simulink model "SeaPort"  (R2023b)
settings: Solver=VariableStepAuto  StartTime=0.0  StopTime=2.0  RelTol=1e-3
(part 1 of 3)
settings Model: Creator=Stefano  LastModifiedBy=stefanopanzieri
settings SolverCC: AlgebraicLoopSolver=TrustRegion
settings OptimizationCC: ReuseModelBlockBuffer=off
settings DebuggingCC: UnconnectedInputMsg=warning  UnconnectedOutputMsg=warning  UnconnectedLineMsg=warning
settings ModelReferenceCC: EnableRefExpFcnMdlSchedulingChecks=on
settings SFSimCC: CustomCodeUndefinedFunction=UseInterfaceOnly
settings RTWCC: DLArmComputeVersion=19.05

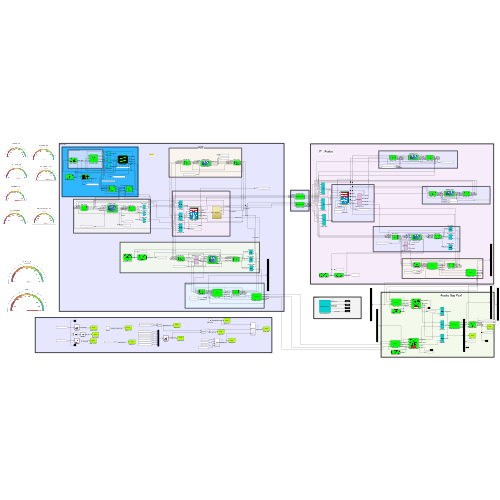
[thumbnail: Simulink's stored preview of the top-level diagram]
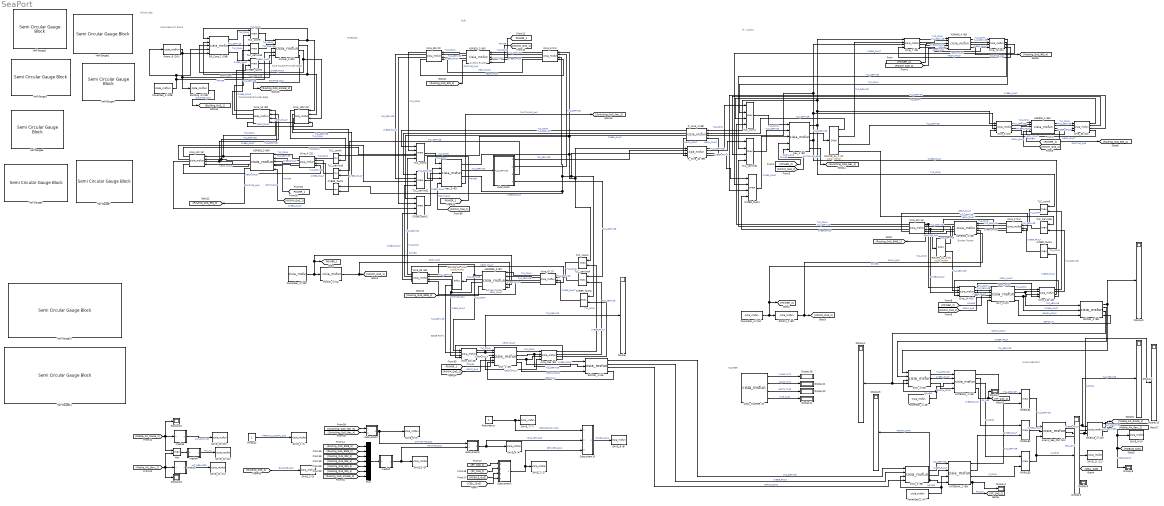
== system SeaPort ==
  note: EDGE POP 1
  note: IT - Aveiro
  note: Altice Labs
  note: CORE DC
  note: Border Router
  note: Access Router
  note: Core Router/Provider Edge
  note: ALB
  note: Aveiro Sea Port
  note: Border Router
  note: Core Network Room
  note: Core Router/Provider Edge
  note: MASTER
  5G_Core_1 (198) : M-S-Function  FunctionName=cisia_msfun  Parameters=Parameter1, Parameter2, Parameter3, resources, Parameter10, codeupdate, step_received, step_computed, dynamic_computed, step_sended, id_entity, id_project, id_type, name_type, color  mask(S-function:msfcn_unit_delay){Parameter1='5G_Core_1', Parameter2=1, Parameter3='ORO', resources=*** INPUT RESOURCES *** NUM_INPUTS 5 TLC_CONN (20) TLC_SERVICE (20) CYBER_FAULT (10) POWER (1) ROOM_QoS (1)  *** STATE VARIABLES *** NUM_VARIABLES 22 Operative_Level(NUMERIC)(1)(1) TLC_services(NUMERIC_ARRAY)(20)(0  0  0  0  0  0  1  1  0  0  0  0  0  0  0  0  0  0  0  0) TLC_service_names(STRING)(100)(5G_CU_DU_SLICE) Connection(NUMERIC_ARRAY)(20)(0  0  0  0  0  0  1  1  0  0  0  0  0  0  0  0  0  0  0  0) Dos_attack(NUMERIC)(1)(0) MITM_attack(NUMERIC)(1)(0) Virus_Attack(NUMERIC)(1)(0) Port_Scan_Attack(NUMERIC)(1)(0) Cyber_Fault(NUMERIC_ARRAY)(10)(0  0  0  0  0  0  0  0  0  0) BGP_hijacking(NUMERIC)(1)(0) Mechanical_Fault(NUMERIC)(1)(0) Conn_Fault(NUMERIC)(1)(0) Consumed_Services(NUMERIC_ARRAY)(20)(0  0  0  0  0  0  0  0  0  0  0  0  0  0  0  0  0  0  0  0) Service_Fault(NUMERIC)(1)(0) Redundancy_Fault(NUMERIC)(1)(0) BotNet_Attack(NUMERIC)(1)(0) Data_Corruption(NUMERIC)(1)(0) syslog_adm_login(NUMERIC)(1)(0) SW_Change(NUMERIC)(1)(0) Config_Change(NUMERIC)(1)(0) Port_Saturation(NUMERIC)(1)(0) TLC_revoke(NUMERIC_ARRAY)(20)(0  0  0  0  0  0  0  0  0  0  0  0  0  0  0  0  0  0  0  0)  *** OUTPUT RESOURCES *** NUM_OUTPUTS 3 TLC_CONN (20) TLC_SERVICE (20) CYBER_FAULT (10), Parameter10=off, codeupdate=off, step_received=Connection=max(Connection_init,TLC_CONN); TLC_services=max(TLC_services_init,TLC_SERVICE); TLC_services=mod(TLC_services,10); TLC_revoke=floor(TLC_SERVICE/10); Mechanical_Fault=max([Mechanical_Fault Mechanical_Fault_init]);  Cyber_Fault=max(CYBER_FAULT, transpose([Dos_attack   MITM_attack Virus_Attack Port_Scan_Attack  BGP_hijacking BotNet_Attack Data_Corruption SW_Change Config_Change Port_Saturation]));    %if (cisia.major_time)>=2    %Dos_attack=1;    %TLC_services(5)=0;   %TLC_revoke(5)=1; %end    Conn_Fault=max([Dos_attack  Mechanical_Fault  1-POWER 1-ROOM_QoS] );  Service_Fault=max(abs(Consumed_Services.*TLC_services-Consumed_Services)); Redundancy_Fault=max(abs(Consumed_Services.*TLC_CONN-Consumed_Services));  Operative_Level=(1-Conn_Fault)*(1-0.5*max(Cyber_Fault))*(1-Service_Fault);, step_computed=, dynamic_computed=, step_sended=TLC_CONN=Connection*(1-Conn_Fault); TLC_SERVICE=TLC_services*(1-Conn_Fault)*(1-Service_Fault)*(1 -syslog_adm_login)+10*TLC_revoke; %TLC_SERVICE=TLC_services CYBER_FAULT=Cyber_Fault*(1-Conn_Fault);, id_entity=198, id_project=40, id_type=38, name_type=5G_Core, color=#E7A6FF}
      mask prompts: Parameter1 "entity name"; Parameter2 "sampling time"; Parameter3 "project"; resources "input resources and state variables"; Parameter10 "Bring state variables to output"; codeupdate "update code from mask"
      mask help: This is a level-2 MATLAB file S-function which demonstrates CISIA entity
      mask DialogControl Container1 Prompt: All parameters
      mask Display: image('Icons/5G_Core.png')
  ANTENNA_1 (56) : M-S-Function  FunctionName=cisia_msfun  Parameters=Parameter1, Parameter2, Parameter3, resources, Parameter10, codeupdate, step_received, step_computed, dynamic_computed, step_sended, id_entity, id_project, id_type, name_type, color  mask(S-function:msfcn_unit_delay){Parameter1='ANTENNA_1', Parameter2=1, Parameter3='ORO', resources=*** INPUT RESOURCES *** NUM_INPUTS 4 TLC_SERVICE (20) CYBER_FAULT (10) POWER (1) NGPON_CONN (20)  *** STATE VARIABLES *** NUM_VARIABLES 20 Operative_Level(NUMERIC)(1)(1) TLC_services(NUMERIC_ARRAY)(20)(0  0  0  0  0  0  0  0  0  0  0  0  0  0  0  0  0  0  0  0) Connection(NUMERIC_ARRAY)(20)(0  0  0  0  0  0  0  0  0  0  0  0  0  0  0  0  0  0  0  0) Dos_attack(NUMERIC)(1)(0) MITM_attack(NUMERIC)(1)(0) Virus_Attack(NUMERIC)(1)(0) Port_Scan_Attack(NUMERIC)(1)(0) Cyber_Fault(NUMERIC_ARRAY)(10)(0  0  0  0  0  0  0  0  0  0) MyConn(NUMERIC_ARRAY)(20)(0  0  0  0  0  0  0  0  0  0  0  0  0  0  0  0  0  0  0  0) BGP_hijacking(NUMERIC)(1)(0) Mechanical_Fault(NUMERIC)(1)(0) Conn_Fault(NUMERIC)(1)(0) Consumed_Services(NUMERIC_ARRAY)(20)(0  0  0  0  0  0  1  0  0  0  0  0  0  0  0  0  0  0  0  0) BotNet_Attack(NUMERIC)(1)(0) Data_Corruption(NUMERIC)(1)(0) SW_Change(NUMERIC)(1)(0) Config_Change(NUMERIC)(1)(0) Port_Saturation(NUMERIC)(1)(0) My_Service(NUMERIC)(1)(0) TLC_revoke(NUMERIC_ARRAY)(20)(0  0  0  0  0  0  0  0  0  0  0  0  0  0  0  0  0  0  0  0)  *** OUTPUT RESOURCES *** NUM_OUTPUTS 4 TLC_SERVICE (20) CYBER_FAULT (10) R_CONN (20) RF_QoS (1), Parameter10=off, codeupdate=off, step_received=Connection=max(Connection_init,NGPON_CONN); TLC_services=max(TLC_services_init,TLC_SERVICE); TLC_services=mod(TLC_services,10); TLC_revoke=floor(TLC_SERVICE/10);  Cyber_Fault=max(CYBER_FAULT, transpose([Dos_attack   MITM_attack Virus_Attack Port_Scan_Attack  BGP_hijacking BotNet_Attack Data_Corruption SW_Change Config_Change Port_Saturation]));  % Vale 1 in presenza di fault Conn_Fault=max([Dos_attack  Mechanical_Fault  1-POWER] );  Service_Fault=max(abs(Consumed_Services.*TLC_services-Consumed_Services)); Redundancy_Fault=max(abs(Consumed_Services.*NGPON_CONN-Consumed_Services));   Operative_Level=(1-Conn_Fault)*max(max(NGPON_CONN),0.5)*((2*(1-Service_Fault)+(1-Redundancy_Fault))/3);  % Il servizio utilizzato My_Service=max([(1-Service_Fault) (1-Redundancy_Fault)/2]);, step_computed=, dynamic_computed=, step_sended=R_CONN=Connection*(1-Conn_Fault); TLC_SERVICE=TLC_services*(1-Conn_Fault)+10*TLC_revoke;  Cyber_Transmitted=min(Cyber_Fault, transpose([0 0 1 0 1 1 0 0 0 1])); CYBER_FAULT=Cyber_Transmitted*(1-Conn_Fault);   RF_QoS=My_Service;, id_entity=56, id_project=40, id_type=13, name_type=RU-DU_ANTENNA, color=#90DB5A}
      mask prompts: Parameter1 "entity name"; Parameter2 "sampling time"; Parameter3 "project"; resources "input resources and state variables"; Parameter10 "Bring state variables to output"; codeupdate "update code from mask"
      mask help: This is a level-2 MATLAB file S-function which demonstrates CISIA entity
      mask DialogControl Container1 Prompt: All parameters
      mask Display: image('Icons/RU-DU_ANTENNA.png')
  ANTENNA_2 (60) : M-S-Function  FunctionName=cisia_msfun  Parameters=Parameter1, Parameter2, Parameter3, resources, Parameter10, codeupdate, step_received, step_computed, dynamic_computed, step_sended, id_entity, id_project, id_type, name_type, color  mask(S-function:msfcn_unit_delay){Parameter1='ANTENNA_2', Parameter2=1, Parameter3='ORO', resources=*** INPUT RESOURCES *** NUM_INPUTS 4 TLC_SERVICE (20) CYBER_FAULT (10) POWER (1) NGPON_CONN (20)  *** STATE VARIABLES *** NUM_VARIABLES 20 Operative_Level(NUMERIC)(1)(1) TLC_services(NUMERIC_ARRAY)(20)(0  0  0  0  0  0  0  0  0  0  0  0  0  0  0  0  0  0  0  0) Connection(NUMERIC_ARRAY)(20)(0  0  0  0  0  0  0  0  0  0  0  0  0  0  0  0  0  0  0  0) Dos_attack(NUMERIC)(1)(0) MITM_attack(NUMERIC)(1)(0) Virus_Attack(NUMERIC)(1)(0) Port_Scan_Attack(NUMERIC)(1)(0) Cyber_Fault(NUMERIC_ARRAY)(10)(0  0  0  0  0  0  0  0  0  0) MyConn(NUMERIC_ARRAY)(20)(0  0  0  0  0  0  0  0  0  0  0  0  0  0  0  0  0  0  0  0) BGP_hijacking(NUMERIC)(1)(0) Mechanical_Fault(NUMERIC)(1)(0) Conn_Fault(NUMERIC)(1)(0) Consumed_Services(NUMERIC_ARRAY)(20)(0  0  0  0  0  0  1  0  0  0  0  0  0  0  0  0  0  0  0  0) BotNet_Attack(NUMERIC)(1)(0) Data_Corruption(NUMERIC)(1)(0) SW_Change(NUMERIC)(1)(0) Config_Change(NUMERIC)(1)(0) Port_Saturation(NUMERIC)(1)(0) My_Service(NUMERIC)(1)(0) TLC_revoke(NUMERIC_ARRAY)(20)(0  0  0  0  0  0  0  0  0  0  0  0  0  0  0  0  0  0  0  0)  *** OUTPUT RESOURCES *** NUM_OUTPUTS 4 TLC_SERVICE (20) CYBER_FAULT (10) R_CONN (20) RF_QoS (1), Parameter10=off, codeupdate=off, step_received=Connection=max(Connection_init,NGPON_CONN); TLC_services=max(TLC_services_init,TLC_SERVICE); TLC_services=mod(TLC_services,10); TLC_revoke=floor(TLC_SERVICE/10);  Cyber_Fault=max(CYBER_FAULT, transpose([Dos_attack   MITM_attack Virus_Attack Port_Scan_Attack  BGP_hijacking BotNet_Attack Data_Corruption SW_Change Config_Change Port_Saturation]));  % Vale 1 in presenza di fault Conn_Fault=max([Dos_attack  Mechanical_Fault  1-POWER] );  Service_Fault=max(abs(Consumed_Services.*TLC_services-Consumed_Services)); Redundancy_Fault=max(abs(Consumed_Services.*NGPON_CONN-Consumed_Services));   Operative_Level=(1-Conn_Fault)*max(max(NGPON_CONN),0.5)*((2*(1-Service_Fault)+(1-Redundancy_Fault))/3);  % Il servizio utilizzato My_Service=max([(1-Service_Fault) (1-Redundancy_Fault)/2]);, step_computed=, dynamic_computed=, step_sended=R_CONN=Connection*(1-Conn_Fault); TLC_SERVICE=TLC_services*(1-Conn_Fault)+10*TLC_revoke;  Cyber_Transmitted=min(Cyber_Fault, transpose([0 0 1 0 1 1 0 0 0 1])); CYBER_FAULT=Cyber_Transmitted*(1-Conn_Fault);   RF_QoS=My_Service;, id_entity=60, id_project=40, id_type=13, name_type=RU-DU_ANTENNA, color=#90DB5A}
      mask prompts: Parameter1 "entity name"; Parameter2 "sampling time"; Parameter3 "project"; resources "input resources and state variables"; Parameter10 "Bring state variables to output"; codeupdate "update code from mask"
      mask help: This is a level-2 MATLAB file S-function which demonstrates CISIA entity
      mask DialogControl Container1 Prompt: All parameters
      mask Display: image('Icons/RU-DU_ANTENNA.png')
  ASR9006_3 (87) : M-S-Function  FunctionName=cisia_msfun  Parameters=Parameter1, Parameter2, Parameter3, resources, Parameter10, codeupdate, step_received, step_computed, dynamic_computed, step_sended, id_entity, id_project, id_type, name_type, color  mask(S-function:msfcn_unit_delay){Parameter1='ASR9006_3', Parameter2=1, Parameter3='ORO', resources=*** INPUT RESOURCES *** NUM_INPUTS 5 TLC_CONN (20) TLC_SERVICE (20) CYBER_FAULT (10) POWER (1) ROOM_QoS (1)  *** STATE VARIABLES *** NUM_VARIABLES 26 Operative_Level(NUMERIC)(1)(1) TLC_services(NUMERIC_ARRAY)(20)(0  0  0  0  0  0  0  0  0  0  0  0  0  0  0  0  0  0  0  0) TLC_service_names(STRING)(100)() Connection(NUMERIC_ARRAY)(20)(0  0  0  0  0  0  0  0  0  0  0  0  0  0  0  0  0  0  0  0) Dos_attack(NUMERIC)(1)(0) MITM_attack(NUMERIC)(1)(0) Virus_Attack(NUMERIC)(1)(0) Port_Scan_Attack(NUMERIC)(1)(0) Cyber_Fault(NUMERIC_ARRAY)(10)(0  0  0  0  0  0  0  0  0  0) BGP_hijacking(NUMERIC)(1)(0) Mechanical_Fault(NUMERIC)(1)(0) Flooding_Fault(NUMERIC)(1)(0) OutboundQoS(NUMERIC)(1)(0) Conn_Fault(NUMERIC)(1)(0) BotNet_Attack(NUMERIC)(1)(0) Data_Corruption(NUMERIC)(1)(0) syslog_adm_login(NUMERIC)(1)(0) SW_Change(NUMERIC)(1)(0) Config_Change(NUMERIC)(1)(0) Port_Saturation(NUMERIC)(1)(0) Congestion_Fault(NUMERIC)(1)(0) Earthquake_Fault(NUMERIC)(1)(0) TLC_revoke(NUMERIC_ARRAY)(20)(0  0  0  0  0  0  0  0  0  0  0  0  0  0  0  0  0  0  0  0) Room_Fault(NUMERIC)(1)(0) Route_Poisoning(NUMERIC)(1)(0) Interface_Down(NUMERIC)(1)(0)  *** OUTPUT RESOURCES *** NUM_OUTPUTS 4 TLC_CONN (20) TLC_SERVICE (20) CYBER_FAULT (10) ROUTING_QoS (1), Parameter10=off, codeupdate=off, step_received=Connection=max(Connection_init,TLC_CONN); TLC_services=max(TLC_services_init,TLC_SERVICE); TLC_services=mod(TLC_services,10); TLC_revoke=floor(TLC_SERVICE/10);  Cyber_Fault=max(CYBER_FAULT, transpose([Dos_attack   MITM_attack Virus_Attack Port_Scan_Attack  BGP_hijacking BotNet_Attack Data_Corruption SW_Change Config_Change Port_Saturation]));   Conn_Fault=max([Dos_attack BGP_hijacking Route_Poisoning Interface_Down Mechanical_Fault  1-POWER 1-ROOM_QoS Earthquake_Fault] );  Room_Fault=1-ROOM_QoS;  Operative_Level=(1-Room_Fault)*(1-Conn_Fault)*max(max(TLC_services),0.5)*(1-0.5*max(Cyber_Fault));, step_computed=, dynamic_computed=, step_sended=TLC_CONN=Connection*(1-Conn_Fault); TLC_SERVICE=TLC_services*(1-Room_Fault)*(1-Conn_Fault)*(1-syslog_adm_login)+10*TLC_revoke;   Cyber_Transmitted=min(Cyber_Fault, transpose([0 0 1 0 1 1 0 0 0 1]));  CYBER_FAULT=Cyber_Transmitted*(1-Conn_Fault);  ROUTING_QoS=Operative_Level;, id_entity=87, id_project=40, id_type=3, name_type=CISCO_router, color=#4DBEEE}
      mask prompts: Parameter1 "entity name"; Parameter2 "sampling time"; Parameter3 "project"; resources "input resources and state variables"; Parameter10 "Bring state variables to output"; codeupdate "update code from mask"
      mask help: This is a level-2 MATLAB file S-function which demonstrates CISIA entity
      mask DialogControl Container1 Prompt: All parameters
      mask Display: image('Icons/CISCO_router.png')
  ASR9006_4 (88) : M-S-Function  FunctionName=cisia_msfun  Parameters=Parameter1, Parameter2, Parameter3, resources, Parameter10, codeupdate, step_received, step_computed, dynamic_computed, step_sended, id_entity, id_project, id_type, name_type, color  mask(S-function:msfcn_unit_delay){Parameter1='ASR9006_4', Parameter2=1, Parameter3='ORO', resources=*** INPUT RESOURCES *** NUM_INPUTS 5 TLC_CONN (20) TLC_SERVICE (20) CYBER_FAULT (10) POWER (1) ROOM_QoS (1)  *** STATE VARIABLES *** NUM_VARIABLES 26 Operative_Level(NUMERIC)(1)(1) TLC_services(NUMERIC_ARRAY)(20)(0  0  0  0  0  0  0  0  0  0  0  0  0  0  0  0  0  0  0  0) TLC_service_names(STRING)(100)() Connection(NUMERIC_ARRAY)(20)(0  0  0  0  0  0  0  0  0  0  0  0  0  0  0  0  0  0  0  0) Dos_attack(NUMERIC)(1)(0) MITM_attack(NUMERIC)(1)(0) Virus_Attack(NUMERIC)(1)(0) Port_Scan_Attack(NUMERIC)(1)(0) Cyber_Fault(NUMERIC_ARRAY)(10)(0  0  0  0  0  0  0  0  0  0) BGP_hijacking(NUMERIC)(1)(0) Mechanical_Fault(NUMERIC)(1)(0) Flooding_Fault(NUMERIC)(1)(0) OutboundQoS(NUMERIC)(1)(0) Conn_Fault(NUMERIC)(1)(0) BotNet_Attack(NUMERIC)(1)(0) Data_Corruption(NUMERIC)(1)(0) syslog_adm_login(NUMERIC)(1)(0) SW_Change(NUMERIC)(1)(0) Config_Change(NUMERIC)(1)(0) Port_Saturation(NUMERIC)(1)(0) Congestion_Fault(NUMERIC)(1)(0) Earthquake_Fault(NUMERIC)(1)(0) TLC_revoke(NUMERIC_ARRAY)(20)(0  0  0  0  0  0  0  0  0  0  0  0  0  0  0  0  0  0  0  0) Room_Fault(NUMERIC)(1)(0) Route_Poisoning(NUMERIC)(1)(0) Interface_Down(NUMERIC)(1)(0)  *** OUTPUT RESOURCES *** NUM_OUTPUTS 4 TLC_CONN (20) TLC_SERVICE (20) CYBER_FAULT (10) ROUTING_QoS (1), Parameter10=off, codeupdate=off, step_received=Connection=max(Connection_init,TLC_CONN); TLC_services=max(TLC_services_init,TLC_SERVICE); TLC_services=mod(TLC_services,10); TLC_revoke=floor(TLC_SERVICE/10);  Cyber_Fault=max(CYBER_FAULT, transpose([Dos_attack   MITM_attack Virus_Attack Port_Scan_Attack  BGP_hijacking BotNet_Attack Data_Corruption SW_Change Config_Change Port_Saturation]));   Conn_Fault=max([Dos_attack BGP_hijacking Route_Poisoning Interface_Down Mechanical_Fault  1-POWER 1-ROOM_QoS Earthquake_Fault] );  Room_Fault=1-ROOM_QoS;  Operative_Level=(1-Room_Fault)*(1-Conn_Fault)*max(max(TLC_services),0.5)*(1-0.5*max(Cyber_Fault));, step_computed=, dynamic_computed=, step_sended=TLC_CONN=Connection*(1-Conn_Fault); TLC_SERVICE=TLC_services*(1-Room_Fault)*(1-Conn_Fault)*(1-syslog_adm_login)+10*TLC_revoke;   Cyber_Transmitted=min(Cyber_Fault, transpose([0 0 1 0 1 1 0 0 0 1]));  CYBER_FAULT=Cyber_Transmitted*(1-Conn_Fault);  ROUTING_QoS=Operative_Level;, id_entity=88, id_project=40, id_type=3, name_type=CISCO_router, color=#4DBEEE}
      mask prompts: Parameter1 "entity name"; Parameter2 "sampling time"; Parameter3 "project"; resources "input resources and state variables"; Parameter10 "Bring state variables to output"; codeupdate "update code from mask"
      mask help: This is a level-2 MATLAB file S-function which demonstrates CISIA entity
      mask DialogControl Container1 Prompt: All parameters
      mask Display: image('Icons/CISCO_router.png')
  ASR903_3 (89) : M-S-Function  FunctionName=cisia_msfun  Parameters=Parameter1, Parameter2, Parameter3, resources, Parameter10, codeupdate, step_received, step_computed, dynamic_computed, step_sended, id_entity, id_project, id_type, name_type, color  mask(S-function:msfcn_unit_delay){Parameter1='ASR903_3', Parameter2=1, Parameter3='ORO', resources=*** INPUT RESOURCES *** NUM_INPUTS 5 TLC_CONN (20) TLC_SERVICE (20) CYBER_FAULT (10) POWER (1) ROOM_QoS (1)  *** STATE VARIABLES *** NUM_VARIABLES 26 Operative_Level(NUMERIC)(1)(1) TLC_services(NUMERIC_ARRAY)(20)(0  0  0  0  0  0  0  0  0  0  0  0  0  0  0  0  0  0  0  0) TLC_service_names(STRING)(100)() Connection(NUMERIC_ARRAY)(20)(0  0  0  0  0  0  0  0  0  0  0  0  0  0  0  0  0  0  0  0) Dos_attack(NUMERIC)(1)(0) MITM_attack(NUMERIC)(1)(0) Virus_Attack(NUMERIC)(1)(0) Port_Scan_Attack(NUMERIC)(1)(0) Cyber_Fault(NUMERIC_ARRAY)(10)(0  0  0  0  0  0  0  0  0  0) BGP_hijacking(NUMERIC)(1)(0) Mechanical_Fault(NUMERIC)(1)(0) Flooding_Fault(NUMERIC)(1)(0) OutboundQoS(NUMERIC)(1)(0) Conn_Fault(NUMERIC)(1)(0) BotNet_Attack(NUMERIC)(1)(0) Data_Corruption(NUMERIC)(1)(0) syslog_adm_login(NUMERIC)(1)(0) SW_Change(NUMERIC)(1)(0) Config_Change(NUMERIC)(1)(0) Port_Saturation(NUMERIC)(1)(0) Congestion_Fault(NUMERIC)(1)(0) Earthquake_Fault(NUMERIC)(1)(0) TLC_revoke(NUMERIC_ARRAY)(20)(0  0  0  0  0  0  0  0  0  0  0  0  0  0  0  0  0  0  0  0) Room_Fault(NUMERIC)(1)(0) Route_Poisoning(NUMERIC)(1)(0) Interface_Down(NUMERIC)(1)(0)  *** OUTPUT RESOURCES *** NUM_OUTPUTS 4 TLC_CONN (20) TLC_SERVICE (20) CYBER_FAULT (10) ROUTING_QoS (1), Parameter10=off, codeupdate=off, step_received=Connection=max(Connection_init,TLC_CONN); TLC_services=max(TLC_services_init,TLC_SERVICE); TLC_services=mod(TLC_services,10); TLC_revoke=floor(TLC_SERVICE/10);  Cyber_Fault=max(CYBER_FAULT, transpose([Dos_attack   MITM_attack Virus_Attack Port_Scan_Attack  BGP_hijacking BotNet_Attack Data_Corruption SW_Change Config_Change Port_Saturation]));   Conn_Fault=max([Dos_attack BGP_hijacking Route_Poisoning Interface_Down Mechanical_Fault  1-POWER 1-ROOM_QoS Earthquake_Fault] );  Room_Fault=1-ROOM_QoS;  Operative_Level=(1-Room_Fault)*(1-Conn_Fault)*max(max(TLC_services),0.5)*(1-0.5*max(Cyber_Fault));, step_computed=, dynamic_computed=, step_sended=TLC_CONN=Connection*(1-Conn_Fault); TLC_SERVICE=TLC_services*(1-Room_Fault)*(1-Conn_Fault)*(1-syslog_adm_login)+10*TLC_revoke;   Cyber_Transmitted=min(Cyber_Fault, transpose([0 0 1 0 1 1 0 0 0 1]));  CYBER_FAULT=Cyber_Transmitted*(1-Conn_Fault);  ROUTING_QoS=Operative_Level;, id_entity=89, id_project=40, id_type=3, name_type=CISCO_router, color=#4DBEEE}
      mask prompts: Parameter1 "entity name"; Parameter2 "sampling time"; Parameter3 "project"; resources "input resources and state variables"; Parameter10 "Bring state variables to output"; codeupdate "update code from mask"
      mask help: This is a level-2 MATLAB file S-function which demonstrates CISIA entity
      mask DialogControl Container1 Prompt: All parameters
      mask Display: image('Icons/CISCO_router.png')
  ASR903_4 (90) : M-S-Function  FunctionName=cisia_msfun  Parameters=Parameter1, Parameter2, Parameter3, resources, Parameter10, codeupdate, step_received, step_computed, dynamic_computed, step_sended, id_entity, id_project, id_type, name_type, color  mask(S-function:msfcn_unit_delay){Parameter1='ASR903_4', Parameter2=1, Parameter3='ORO', resources=*** INPUT RESOURCES *** NUM_INPUTS 5 TLC_CONN (20) TLC_SERVICE (20) CYBER_FAULT (10) POWER (1) ROOM_QoS (1)  *** STATE VARIABLES *** NUM_VARIABLES 26 Operative_Level(NUMERIC)(1)(1) TLC_services(NUMERIC_ARRAY)(20)(0  0  0  0  0  0  0  0  0  0  0  0  0  0  0  0  0  0  0  0) TLC_service_names(STRING)(100)() Connection(NUMERIC_ARRAY)(20)(0  0  0  0  0  0  0  0  0  0  0  0  0  0  0  0  0  0  0  0) Dos_attack(NUMERIC)(1)(0) MITM_attack(NUMERIC)(1)(0) Virus_Attack(NUMERIC)(1)(0) Port_Scan_Attack(NUMERIC)(1)(0) Cyber_Fault(NUMERIC_ARRAY)(10)(0  0  0  0  0  0  0  0  0  0) BGP_hijacking(NUMERIC)(1)(0) Mechanical_Fault(NUMERIC)(1)(0) Flooding_Fault(NUMERIC)(1)(0) OutboundQoS(NUMERIC)(1)(0) Conn_Fault(NUMERIC)(1)(0) BotNet_Attack(NUMERIC)(1)(0) Data_Corruption(NUMERIC)(1)(0) syslog_adm_login(NUMERIC)(1)(0) SW_Change(NUMERIC)(1)(0) Config_Change(NUMERIC)(1)(0) Port_Saturation(NUMERIC)(1)(0) Congestion_Fault(NUMERIC)(1)(0) Earthquake_Fault(NUMERIC)(1)(0) TLC_revoke(NUMERIC_ARRAY)(20)(0  0  0  0  0  0  0  0  0  0  0  0  0  0  0  0  0  0  0  0) Room_Fault(NUMERIC)(1)(0) Route_Poisoning(NUMERIC)(1)(0) Interface_Down(NUMERIC)(1)(0)  *** OUTPUT RESOURCES *** NUM_OUTPUTS 4 TLC_CONN (20) TLC_SERVICE (20) CYBER_FAULT (10) ROUTING_QoS (1), Parameter10=off, codeupdate=off, step_received=Connection=max(Connection_init,TLC_CONN); TLC_services=max(TLC_services_init,TLC_SERVICE); TLC_services=mod(TLC_services,10); TLC_revoke=floor(TLC_SERVICE/10);  Cyber_Fault=max(CYBER_FAULT, transpose([Dos_attack   MITM_attack Virus_Attack Port_Scan_Attack  BGP_hijacking BotNet_Attack Data_Corruption SW_Change Config_Change Port_Saturation]));   Conn_Fault=max([Dos_attack BGP_hijacking Route_Poisoning Interface_Down Mechanical_Fault  1-POWER 1-ROOM_QoS Earthquake_Fault] );  Room_Fault=1-ROOM_QoS;  Operative_Level=(1-Room_Fault)*(1-Conn_Fault)*max(max(TLC_services),0.5)*(1-0.5*max(Cyber_Fault));, step_computed=, dynamic_computed=, step_sended=TLC_CONN=Connection*(1-Conn_Fault); TLC_SERVICE=TLC_services*(1-Room_Fault)*(1-Conn_Fault)*(1-syslog_adm_login)+10*TLC_revoke;   Cyber_Transmitted=min(Cyber_Fault, transpose([0 0 1 0 1 1 0 0 0 1]));  CYBER_FAULT=Cyber_Transmitted*(1-Conn_Fault);  ROUTING_QoS=Operative_Level;, id_entity=90, id_project=40, id_type=3, name_type=CISCO_router, color=#4DBEEE}
      mask prompts: Parameter1 "entity name"; Parameter2 "sampling time"; Parameter3 "project"; resources "input resources and state variables"; Parameter10 "Bring state variables to output"; codeupdate "update code from mask"
      mask help: This is a level-2 MATLAB file S-function which demonstrates CISIA entity
      mask DialogControl Container1 Prompt: All parameters
      mask Display: image('Icons/CISCO_router.png')
  ASR920_3 (85) : M-S-Function  FunctionName=cisia_msfun  Parameters=Parameter1, Parameter2, Parameter3, resources, Parameter10, codeupdate, step_received, step_computed, dynamic_computed, step_sended, id_entity, id_project, id_type, name_type, color  mask(S-function:msfcn_unit_delay){Parameter1='ASR920_3', Parameter2=1, Parameter3='ORO', resources=*** INPUT RESOURCES *** NUM_INPUTS 5 TLC_CONN (20) TLC_SERVICE (20) CYBER_FAULT (10) POWER (1) ROOM_QoS (1)  *** STATE VARIABLES *** NUM_VARIABLES 26 Operative_Level(NUMERIC)(1)(1) TLC_services(NUMERIC_ARRAY)(20)(0  0  0  0  0  0  0  0  0  0  0  0  0  0  0  0  0  0  0  0) TLC_service_names(STRING)(100)() Connection(NUMERIC_ARRAY)(20)(0  0  0  0  0  0  0  0  0  0  0  0  0  0  0  0  0  0  0  0) Dos_attack(NUMERIC)(1)(0) MITM_attack(NUMERIC)(1)(0) Virus_Attack(NUMERIC)(1)(0) Port_Scan_Attack(NUMERIC)(1)(0) Cyber_Fault(NUMERIC_ARRAY)(10)(0  0  0  0  0  0  0  0  0  0) BGP_hijacking(NUMERIC)(1)(0) Mechanical_Fault(NUMERIC)(1)(0) Flooding_Fault(NUMERIC)(1)(0) OutboundQoS(NUMERIC)(1)(0) Conn_Fault(NUMERIC)(1)(0) BotNet_Attack(NUMERIC)(1)(0) Data_Corruption(NUMERIC)(1)(0) syslog_adm_login(NUMERIC)(1)(0) SW_Change(NUMERIC)(1)(0) Config_Change(NUMERIC)(1)(0) Port_Saturation(NUMERIC)(1)(0) Congestion_Fault(NUMERIC)(1)(0) Earthquake_Fault(NUMERIC)(1)(0) TLC_revoke(NUMERIC_ARRAY)(20)(0  0  0  0  0  0  0  0  0  0  0  0  0  0  0  0  0  0  0  0) Room_Fault(NUMERIC)(1)(0) Route_Poisoning(NUMERIC)(1)(0) Interface_Down(NUMERIC)(1)(0)  *** OUTPUT RESOURCES *** NUM_OUTPUTS 4 TLC_CONN (20) TLC_SERVICE (20) CYBER_FAULT (10) ROUTING_QoS (1), Parameter10=off, codeupdate=off, step_received=Connection=max(Connection_init,TLC_CONN); TLC_services=max(TLC_services_init,TLC_SERVICE); TLC_services=mod(TLC_services,10); TLC_revoke=floor(TLC_SERVICE/10);  Cyber_Fault=max(CYBER_FAULT, transpose([Dos_attack   MITM_attack Virus_Attack Port_Scan_Attack  BGP_hijacking BotNet_Attack Data_Corruption SW_Change Config_Change Port_Saturation]));   Conn_Fault=max([Dos_attack BGP_hijacking Route_Poisoning Interface_Down Mechanical_Fault  1-POWER 1-ROOM_QoS Earthquake_Fault] );  Room_Fault=1-ROOM_QoS;  Operative_Level=(1-Room_Fault)*(1-Conn_Fault)*max(max(TLC_services),0.5)*(1-0.5*max(Cyber_Fault));, step_computed=, dynamic_computed=, step_sended=TLC_CONN=Connection*(1-Conn_Fault); TLC_SERVICE=TLC_services*(1-Room_Fault)*(1-Conn_Fault)*(1-syslog_adm_login)+10*TLC_revoke;   Cyber_Transmitted=min(Cyber_Fault, transpose([0 0 1 0 1 1 0 0 0 1]));  CYBER_FAULT=Cyber_Transmitted*(1-Conn_Fault);  ROUTING_QoS=Operative_Level;, id_entity=85, id_project=40, id_type=3, name_type=CISCO_router, color=#4DBEEE}
      mask prompts: Parameter1 "entity name"; Parameter2 "sampling time"; Parameter3 "project"; resources "input resources and state variables"; Parameter10 "Bring state variables to output"; codeupdate "update code from mask"
      mask help: This is a level-2 MATLAB file S-function which demonstrates CISIA entity
      mask DialogControl Container1 Prompt: All parameters
      mask Display: image('Icons/CISCO_router.png')
  ASR920_4 (86) : M-S-Function  FunctionName=cisia_msfun  Parameters=Parameter1, Parameter2, Parameter3, resources, Parameter10, codeupdate, step_received, step_computed, dynamic_computed, step_sended, id_entity, id_project, id_type, name_type, color  mask(S-function:msfcn_unit_delay){Parameter1='ASR920_4', Parameter2=1, Parameter3='ORO', resources=*** INPUT RESOURCES *** NUM_INPUTS 5 TLC_CONN (20) TLC_SERVICE (20) CYBER_FAULT (10) POWER (1) ROOM_QoS (1)  *** STATE VARIABLES *** NUM_VARIABLES 26 Operative_Level(NUMERIC)(1)(1) TLC_services(NUMERIC_ARRAY)(20)(0  0  0  0  0  0  0  0  0  0  0  0  0  0  0  0  0  0  0  0) TLC_service_names(STRING)(100)() Connection(NUMERIC_ARRAY)(20)(0  0  0  0  0  0  0  0  0  0  0  0  0  0  0  0  0  0  0  0) Dos_attack(NUMERIC)(1)(0) MITM_attack(NUMERIC)(1)(0) Virus_Attack(NUMERIC)(1)(0) Port_Scan_Attack(NUMERIC)(1)(0) Cyber_Fault(NUMERIC_ARRAY)(10)(0  0  0  0  0  0  0  0  0  0) BGP_hijacking(NUMERIC)(1)(0) Mechanical_Fault(NUMERIC)(1)(0) Flooding_Fault(NUMERIC)(1)(0) OutboundQoS(NUMERIC)(1)(0) Conn_Fault(NUMERIC)(1)(0) BotNet_Attack(NUMERIC)(1)(0) Data_Corruption(NUMERIC)(1)(0) syslog_adm_login(NUMERIC)(1)(0) SW_Change(NUMERIC)(1)(0) Config_Change(NUMERIC)(1)(0) Port_Saturation(NUMERIC)(1)(0) Congestion_Fault(NUMERIC)(1)(0) Earthquake_Fault(NUMERIC)(1)(0) TLC_revoke(NUMERIC_ARRAY)(20)(0  0  0  0  0  0  0  0  0  0  0  0  0  0  0  0  0  0  0  0) Room_Fault(NUMERIC)(1)(0) Route_Poisoning(NUMERIC)(1)(0) Interface_Down(NUMERIC)(1)(0)  *** OUTPUT RESOURCES *** NUM_OUTPUTS 4 TLC_CONN (20) TLC_SERVICE (20) CYBER_FAULT (10) ROUTING_QoS (1), Parameter10=off, codeupdate=off, step_received=Connection=max(Connection_init,TLC_CONN); TLC_services=max(TLC_services_init,TLC_SERVICE); TLC_services=mod(TLC_services,10); TLC_revoke=floor(TLC_SERVICE/10);  Cyber_Fault=max(CYBER_FAULT, transpose([Dos_attack   MITM_attack Virus_Attack Port_Scan_Attack  BGP_hijacking BotNet_Attack Data_Corruption SW_Change Config_Change Port_Saturation]));   Conn_Fault=max([Dos_attack BGP_hijacking Route_Poisoning Interface_Down Mechanical_Fault  1-POWER 1-ROOM_QoS Earthquake_Fault] );  Room_Fault=1-ROOM_QoS;  Operative_Level=(1-Room_Fault)*(1-Conn_Fault)*max(max(TLC_services),0.5)*(1-0.5*max(Cyber_Fault));, step_computed=, dynamic_computed=, step_sended=TLC_CONN=Connection*(1-Conn_Fault); TLC_SERVICE=TLC_services*(1-Room_Fault)*(1-Conn_Fault)*(1-syslog_adm_login)+10*TLC_revoke;   Cyber_Transmitted=min(Cyber_Fault, transpose([0 0 1 0 1 1 0 0 0 1]));  CYBER_FAULT=Cyber_Transmitted*(1-Conn_Fault);  ROUTING_QoS=Operative_Level;, id_entity=86, id_project=40, id_type=3, name_type=CISCO_router, color=#4DBEEE}
      mask prompts: Parameter1 "entity name"; Parameter2 "sampling time"; Parameter3 "project"; resources "input resources and state variables"; Parameter10 "Bring state variables to output"; codeupdate "update code from mask"
      mask help: This is a level-2 MATLAB file S-function which demonstrates CISIA entity
      mask DialogControl Container1 Prompt: All parameters
      mask Display: image('Icons/CISCO_router.png')
  Alcatel_3 (83) : M-S-Function  FunctionName=cisia_msfun  Parameters=Parameter1, Parameter2, Parameter3, resources, Parameter10, codeupdate, step_received, step_computed, dynamic_computed, step_sended, id_entity, id_project, id_type, name_type, color  mask(S-function:msfcn_unit_delay){Parameter1='Alcatel_3', Parameter2=1, Parameter3='ORO', resources=*** INPUT RESOURCES *** NUM_INPUTS 5 TLC_CONN (20) TLC_SERVICE (20) CYBER_FAULT (10) POWER (1) ROOM_QoS (1)  *** STATE VARIABLES *** NUM_VARIABLES 18 Operative_Level(NUMERIC)(1)(1) TLC_services(NUMERIC_ARRAY)(20)(0  0  0  0  0  0  0  0  0  0  0  0  0  0  0  0  0  0  0  0) TLC_service_names(STRING)(100)() Connection(NUMERIC_ARRAY)(20)(0  0  0  0  0  0  0  0  0  0  0  0  0  0  0  0  0  0  0  0) Dos_attack(NUMERIC)(1)(0) MITM_attack(NUMERIC)(1)(0) Virus_Attack(NUMERIC)(1)(0) Port_Scan_Attack(NUMERIC)(1)(0) Cyber_Fault(NUMERIC_ARRAY)(10)(0  0  0  0  0  0  0  0  0  0) BGP_hijacking(NUMERIC)(1)(0) Mechanical_Fault(NUMERIC)(1)(0) Conn_Fault(NUMERIC)(1)(0) BotNet_Attack(NUMERIC)(1)(0) Data_Corruption(NUMERIC)(1)(0) SW_Change(NUMERIC)(1)(0) Config_Change(NUMERIC)(1)(0) Port_Saturation(NUMERIC)(1)(0) TLC_revoke(NUMERIC_ARRAY)(20)(0  0  0  0  0  0  0  0  0  0  0  0  0  0  0  0  0  0  0  0)  *** OUTPUT RESOURCES *** NUM_OUTPUTS 4 TLC_CONN (20) TLC_SERVICE (20) CYBER_FAULT (10) ROUTING_QoS (1), Parameter10=off, codeupdate=off, step_received=Connection=max(Connection_init,TLC_CONN); TLC_services=max(TLC_services_init,TLC_SERVICE); TLC_services=mod(TLC_services,10); TLC_revoke=floor(TLC_SERVICE/10);  Cyber_Fault=max(CYBER_FAULT, transpose([Dos_attack   MITM_attack Virus_Attack Port_Scan_Attack  BGP_hijacking BotNet_Attack Data_Corruption SW_Change Config_Change Port_Saturation]));  Conn_Fault=max([Dos_attack  Mechanical_Fault  1-POWER 1-ROOM_QoS] );   Operative_Level=(1-Conn_Fault)*(1-0.5*max(Cyber_Fault))*max(max(TLC_services),0.5);, step_computed=, dynamic_computed=, step_sended=TLC_CONN=Connection*(1-Conn_Fault); TLC_SERVICE=TLC_services*(1-Conn_Fault)+TLC_revoke*10; CYBER_FAULT=Cyber_Fault*(1-Conn_Fault);  ROUTING_QoS=Operative_Level;, id_entity=83, id_project=40, id_type=5, name_type=Alcatel7750, color=#ACBD7E}
      mask prompts: Parameter1 "entity name"; Parameter2 "sampling time"; Parameter3 "project"; resources "input resources and state variables"; Parameter10 "Bring state variables to output"; codeupdate "update code from mask"
      mask help: This is a level-2 MATLAB file S-function which demonstrates CISIA entity
      mask DialogControl Container1 Prompt: All parameters
      mask Display: image('Icons/Alcatel7750.png')
  Aveiro_Sea_Port (61) : M-S-Function  FunctionName=cisia_msfun  Parameters=Parameter1, Parameter2, Parameter3, resources, Parameter10, codeupdate, step_received, step_computed, dynamic_computed, step_sended, id_entity, id_project, id_type, name_type, color  mask(S-function:msfcn_unit_delay){Parameter1='Aveiro_Sea_Port', Parameter2=1, Parameter3='ORO', resources=*** INPUT RESOURCES *** NUM_INPUTS 3 TLC_SERVICE (20) CYBER_FAULT (10) R_CONN (20)  *** STATE VARIABLES *** NUM_VARIABLES 25 Operative_Level(NUMERIC)(1)(1) TLC_services(NUMERIC_ARRAY)(20)(0  0  0  0  0  0  0  0  0  0  0  0  0  0  0  0  0  0  0  0) Connection(NUMERIC_ARRAY)(20)(0  0  0  0  0  0  0  0  0  0  0  0  0  0  0  0  0  0  0  0) Dos_attack(NUMERIC)(1)(0) MITM_attack(NUMERIC)(1)(0) Virus_Attack(NUMERIC)(1)(0) Port_Scan_Attack(NUMERIC)(1)(0) Cyber_Fault(NUMERIC_ARRAY)(10)(0  0  0  0  0  0  0  0  0  0) BGP_hijacking(NUMERIC)(1)(0) Mechanical_Fault(NUMERIC)(1)(0) Unauthorized_Access(NUMERIC)(1)(0) Conn_Fault(NUMERIC)(1)(0) Consumed_Services(NUMERIC_ARRAY)(20)(0  0  0  0  0  0  1  1  0  0  0  0  0  0  0  0  0  0  0  0) Service_Fault(NUMERIC)(1)(0) Redundancy_Fault(NUMERIC)(1)(0) BotNet_Attack(NUMERIC)(1)(0) Data_Corruption(NUMERIC)(1)(0) Rouge_Access(NUMERIC)(1)(0) SW_Change(NUMERIC)(1)(0) Config_Change(NUMERIC)(1)(0) Port_Saturation(NUMERIC)(1)(0) Perimeter_Security_Fault(NUMERIC)(1)(0) Security_Camera_Fault(NUMERIC)(1)(0) My_Service(NUMERIC)(1)(0) TLC_revoke(NUMERIC_ARRAY)(20)(0  0  0  0  0  0  0  0  0  0  0  0  0  0  0  0  0  0  0  0)  *** OUTPUT RESOURCES *** NUM_OUTPUTS 4 TLC_SERVICE (20) CYBER_FAULT (10) R_CONN (20) CELL_QoS (1), Parameter10=off, codeupdate=off, step_received=Connection=max(Connection_init,R_CONN); TLC_services=max(TLC_services_init,TLC_SERVICE); TLC_services=mod(TLC_services,10); TLC_revoke=floor(TLC_SERVICE/10);  Cyber_Fault=max(CYBER_FAULT, transpose([Dos_attack   MITM_attack Virus_Attack Port_Scan_Attack  BGP_hijacking BotNet_Attack Data_Corruption SW_Change Config_Change Port_Saturation]));  % Vale 1 in presenza di fault Conn_Fault=max([Dos_attack  Mechanical_Fault] );  Service_Fault=max(abs(Consumed_Services.*TLC_services-Consumed_Services)); Redundancy_Fault=max(abs(Consumed_Services.*R_CONN-Consumed_Services));   Operative_Level=(1-Conn_Fault)*max(max(R_CONN),0.5)*((2*(1-Service_Fault)+(1-Redundancy_Fault))/3);  % Il servizio utilizzato My_Service=max([(1-Service_Fault) (1-Redundancy_Fault)/2]);, step_computed=, dynamic_computed=, step_sended=R_CONN=Connection*(1-Conn_Fault); TLC_SERVICE=TLC_services*(1-Conn_Fault)+10*TLC_revoke; CYBER_FAULT=Cyber_Fault*(1-Conn_Fault);  CELL_QoS=My_Service;, id_entity=61, id_project=40, id_type=14, name_type=Cell_Area, color=#0FFFFF}
      mask prompts: Parameter1 "entity name"; Parameter2 "sampling time"; Parameter3 "project"; resources "input resources and state variables"; Parameter10 "Bring state variables to output"; codeupdate "update code from mask"
      mask help: This is a level-2 MATLAB file S-function which demonstrates CISIA entity
      mask DialogControl Container1 Prompt: All parameters
      mask Display: disp('Cell_Area')
  Building_3 (215) : M-S-Function  FunctionName=cisia_msfun  Parameters=Parameter1, Parameter2, Parameter3, resources, Parameter10, codeupdate, step_received, step_computed, dynamic_computed, step_sended, id_entity, id_project, id_type, name_type, color  mask(S-function:msfcn_unit_delay){Parameter1='Building_3', Parameter2=1, Parameter3='ORO', resources=*** INPUT RESOURCES *** NUM_INPUTS 1 ROOM_QoS (1)  *** STATE VARIABLES *** NUM_VARIABLES 9 Operative_Level(NUMERIC)(1)(1) Cyber_Fault(NUMERIC_ARRAY)(10)(0  0  0  0  0  0  0  0  0  0) Power_Fault(NUMERIC)(1)(0) Unauthorized_Access(NUMERIC)(1)(0) Conn_Fault(NUMERIC)(1)(0) Perimeter_Security_Fault(NUMERIC)(1)(0) Security_Camera_Fault(NUMERIC)(1)(0) Earthquake_Fault(NUMERIC)(1)(0) Physical_Fault(NUMERIC)(1)(0)  *** OUTPUT RESOURCES *** NUM_OUTPUTS 2 CYBER_FAULT (10) BUILDING_QoS (1), Parameter10=off, codeupdate=off, step_received=Physical_Fault=max([Unauthorized_Access Perimeter_Security_Fault Security_Camera_Fault Earthquake_Fault]);  Conn_Fault=max([Power_Fault 1-ROOM_QoS]);  Operative_Level=min([ (1-Physical_Fault) (1-Conn_Fault) (1-Perimeter_Security_Fault) (1-Earthquake_Fault) ]);, step_computed=, dynamic_computed=, step_sended=BUILDING_QoS=Operative_Level;  %Cyber_Fault=0.3*ones(size(Cyber_Fault));  CYBER_FAULT=Perimeter_Security_Fault*Cyber_Fault;, id_entity=215, id_project=40, id_type=10, name_type=Building, color=#AB7A07}
      mask prompts: Parameter1 "entity name"; Parameter2 "sampling time"; Parameter3 "project"; resources "input resources and state variables"; Parameter10 "Bring state variables to output"; codeupdate "update code from mask"
      mask help: This is a level-2 MATLAB file S-function which demonstrates CISIA entity
      mask DialogControl Container1 Prompt: All parameters
      mask Display: image('Icons/Building.png')
  CISIA_MASTER (0) : M-S-Function  FunctionName=cisia_msfun  Parameters=Parameter1, Parameter2, Parameter3, resources, Parameter4, Parameter5, Parameter6, Parameter7, Parameter8, Parameter9,Parameter11,Parameter12  mask(S-function:msfcn_unit_delay){Parameter1='CISIA_MASTER', Parameter2=[1], Parameter3='SeaPort', resources=off, Parameter4=on, Parameter5=off, Parameter6=off, Parameter7=off, Parameter8=0.001, Parameter9=off, Parameter11=on, Parameter12=off}
      mask prompts: Parameter1 "entity name"; Parameter2 "sampling time"; Parameter3 "project"; resources "Save status at each major hit"; Parameter4 "Show Operative Levels with colors"; Parameter5 "Load Entities from file"; Parameter6 "Load Start from Mask"; Parameter7 "Real Time"; Parameter8 "Real Time Hit (sec)"; Parameter9 "Skip saving"; Parameter11 "Show unconnected"; Parameter12 "Save port values"
      mask help: MASTER BLOCK v.2.0
      mask Display: disp('MASTER BLOCK')
  CYBER_fault{1,3..4,9} (4 alike) : MinMax  Function=max  Inputs=2
  "CYBER_fault1 " : MinMax  Function=max  Inputs=4
  CYBER_fault2 : MinMax  Function=max  Inputs=4
  Display{,1..11,15..16,18,20..21} (17 alike) : Display
  Firewall : Constant
  Half Gauge{1..5,7..8,10..11} (9 alike) : SemiCircularGaugeBlock  ScaleMax=1
  MOBILE1 : MinMax  Function=max  Inputs=2
  MOBILE2 : MinMax  Function=max  Inputs=2
  MOBILE3 : MinMax  Function=max  Inputs=2
  MOBILE_1 (147) : M-S-Function  FunctionName=cisia_msfun  Parameters=Parameter1, Parameter2, Parameter3, resources, Parameter10, codeupdate, step_received, step_computed, dynamic_computed, step_sended, id_entity, id_project, id_type, name_type, color  mask(S-function:msfcn_unit_delay){Parameter1='MOBILE_1', Parameter2=1, Parameter3='ORO', resources=*** INPUT RESOURCES *** NUM_INPUTS 3 TLC_SERVICE (20) CYBER_FAULT (10) R_CONN (20)  *** STATE VARIABLES *** NUM_VARIABLES 26 Operative_Level(NUMERIC)(1)(1) TLC_services(NUMERIC_ARRAY)(20)(0  0  0  0  0  0  0  0  0  0  0  0  0  0  0  0  0  0  0  0) Connection(NUMERIC_ARRAY)(20)(0  0  0  0  0  0  0  0  0  0  0  0  0  0  0  0  0  0  0  0) Dos_attack(NUMERIC)(1)(0) MITM_attack(NUMERIC)(1)(0) Virus_Attack(NUMERIC)(1)(0) Port_Scan_Attack(NUMERIC)(1)(0) Cyber_Fault(NUMERIC_ARRAY)(10)(0  0  0  0  0  0  0  0  0  0) BGP_hijacking(NUMERIC)(1)(0) Mechanical_Fault(NUMERIC)(1)(0) Conn_Fault(NUMERIC)(1)(0) Consumed_Services(NUMERIC_ARRAY)(20)(0  0  0  0  0  0  1  1  0  0  0  0  0  0  0  0  0  0  0  0) Service_Fault(NUMERIC)(1)(0) Redundancy_Fault(NUMERIC)(1)(0) BotNet_Attack(NUMERIC)(1)(0) Data_Corruption(NUMERIC)(1)(0) SW_Change(NUMERIC)(1)(0) Config_Change(NUMERIC)(1)(0) Port_Saturation(NUMERIC)(1)(0) My_Service(NUMERIC)(1)(0) TLC_revoke(NUMERIC_ARRAY)(20)(0  0  0  0  0  0  0  0  0  0  0  0  0  0  0  0  0  0  0  0) Alternative_Services(NUMERIC_ARRAY)(20)(1  1  0  0  0  0  0  0  0  0  0  0  0  0  0  0  0  0  0  0) Alt_Serv_Fault(NUMERIC)(1)(0) Alt_Rout_Fault(NUMERIC)(1)(0) Port_Isolation(NUMERIC)(1)(0) Alt_Port_Isol(NUMERIC)(1)(0)  *** OUTPUT RESOURCES *** NUM_OUTPUTS 4 MOBILE_QoS (1) ALT_ROUTING (1) ALT_SERVICES (1) ALT_PORT_ISOLATION (1), Parameter10=off, codeupdate=off, step_received=Connection=max(Connection_init,R_CONN); TLC_services=max(TLC_services_init,TLC_SERVICE); TLC_services=mod(TLC_services,10); TLC_revoke=floor(TLC_SERVICE/10);  Service_Fault=max(abs(Consumed_Services.*TLC_services-Consumed_Services)); Redundancy_Fault=max(abs(Consumed_Services.*R_CONN-Consumed_Services));  Alt_Serv_Fault=max(abs(Alternative_Services.*R_CONN-Alternative_Services));  Alt_Rout_Fault=max(abs(Consumed_Services.*R_CONN-Consumed_Services));  Port_Isolation=min(max(transpose([1 1 1 1 1 1 1 1 1 0]), CYBER_FAULT));   Operative_Level=(1-Mechanical_Fault)*max(max(R_CONN), 0.5)*(((1-Service_Fault)+(1-Redundancy_Fault)+(1-Port_Isolation))/3);  Alt_Port_Isol=(1-Mechanical_Fault)*max(max(R_CONN), 0.5)*(((1-Service_Fault)+(1-Redundancy_Fault))/2);, step_computed=, dynamic_computed=, step_sended=MOBILE_QoS=Operative_Level;   ALT_SERVICES=1-Alt_Serv_Fault; ALT_ROUTING=1-Alt_Rout_Fault; ALT_PORT_ISOLATION=Alt_Port_Isol;, id_entity=147, id_project=40, id_type=39, name_type=MobileUnit, color=#C9ABDB}
      mask prompts: Parameter1 "entity name"; Parameter2 "sampling time"; Parameter3 "project"; resources "input resources and state variables"; Parameter10 "Bring state variables to output"; codeupdate "update code from mask"
      mask help: This is a level-2 MATLAB file S-function which demonstrates CISIA entity
      mask DialogControl Container1 Prompt: All parameters
      mask Display: image('Icons/MobileUnit.png')
  Max : MinMax  Function=max  Inputs=2
  Mux : Mux  Inputs=7
  Nex_3 (92) : M-S-Function  FunctionName=cisia_msfun  Parameters=Parameter1, Parameter2, Parameter3, resources, Parameter10, codeupdate, step_received, step_computed, dynamic_computed, step_sended, id_entity, id_project, id_type, name_type, color  mask(S-function:msfcn_unit_delay){Parameter1='Nex_3', Parameter2=1, Parameter3='ORO', resources=*** INPUT RESOURCES *** NUM_INPUTS 5 TLC_CONN (20) TLC_SERVICE (20) CYBER_FAULT (10) POWER (1) ROOM_QoS (1)  *** STATE VARIABLES *** NUM_VARIABLES 17 Operative_Level(NUMERIC)(1)(1) TLC_services(NUMERIC_ARRAY)(20)(0  0  0  0  0  0  0  0  0  0  0  0  0  0  0  0  0  0  0  0) Connection(NUMERIC_ARRAY)(20)(0  0  0  0  0  0  0  0  0  0  0  0  0  0  0  0  0  0  0  0) Dos_attack(NUMERIC)(1)(0) MITM_attack(NUMERIC)(1)(0) Virus_Attack(NUMERIC)(1)(0) Port_Scan_Attack(NUMERIC)(1)(0) Cyber_Fault(NUMERIC_ARRAY)(10)(0  0  0  0  0  0  0  0  0  0) BGP_hijacking(NUMERIC)(1)(0) Mechanical_Fault(NUMERIC)(1)(0) Conn_Fault(NUMERIC)(1)(0) BotNet_Attack(NUMERIC)(1)(0) Data_Corruption(NUMERIC)(1)(0) SW_Change(NUMERIC)(1)(0) Config_Change(NUMERIC)(1)(0) Port_Saturation(NUMERIC)(1)(0) TLC_revoke(NUMERIC_ARRAY)(20)(0  0  0  0  0  0  0  0  0  0  0  0  0  0  0  0  0  0  0  0)  *** OUTPUT RESOURCES *** NUM_OUTPUTS 4 TLC_CONN (20) TLC_SERVICE (20) CYBER_FAULT (10) SWITCHING_QoS (1), Parameter10=off, codeupdate=off, step_received=Connection=max(Connection_init,TLC_CONN);  TLC_services=max(TLC_services_init,TLC_SERVICE); TLC_services=mod(TLC_services,10); TLC_revoke=floor(TLC_SERVICE/10);  Cyber_Fault=max(CYBER_FAULT, transpose([Dos_attack   MITM_attack Virus_Attack Port_Scan_Attack  BGP_hijacking BotNet_Attack Data_Corruption SW_Change Config_Change Port_Saturation]));  Conn_Fault=max([Dos_attack  Mechanical_Fault  1-POWER 1-ROOM_QoS] );  Operative_Level=(1-Conn_Fault)*max(max(TLC_services),0.5)*(1-0.5*max(Cyber_Fault));, step_computed=, dynamic_computed=, step_sended=TLC_CONN=Connection*(1-Conn_Fault); TLC_SERVICE=TLC_services*(1-Conn_Fault)+10*TLC_revoke;  Cyber_Transmitted=min(Cyber_Fault, transpose([0 0 1 0 1 1 0 0 0 1])); CYBER_FAULT=Cyber_Transmitted*(1-Conn_Fault);   SWITCHING_QoS=Operative_Level;, id_entity=92, id_project=40, id_type=2, name_type=Nexus93180Switch, color=#0072BD}
      mask prompts: Parameter1 "entity name"; Parameter2 "sampling time"; Parameter3 "project"; resources "input resources and state variables"; Parameter10 "Bring state variables to output"; codeupdate "update code from mask"
      mask help: This is a level-2 MATLAB file S-function which demonstrates CISIA entity
      mask DialogControl Container1 Prompt: All parameters
      mask Display: image('Icons/Nexus93180Switch.png')
  Nex_4 (93) : M-S-Function  FunctionName=cisia_msfun  Parameters=Parameter1, Parameter2, Parameter3, resources, Parameter10, codeupdate, step_received, step_computed, dynamic_computed, step_sended, id_entity, id_project, id_type, name_type, color  mask(S-function:msfcn_unit_delay){Parameter1='Nex_4', Parameter2=1, Parameter3='ORO', resources=*** INPUT RESOURCES *** NUM_INPUTS 5 TLC_CONN (20) TLC_SERVICE (20) CYBER_FAULT (10) POWER (1) ROOM_QoS (1)  *** STATE VARIABLES *** NUM_VARIABLES 17 Operative_Level(NUMERIC)(1)(1) TLC_services(NUMERIC_ARRAY)(20)(0  0  0  0  0  0  0  0  0  0  0  0  0  0  0  0  0  0  0  0) Connection(NUMERIC_ARRAY)(20)(0  0  0  0  0  0  0  0  0  0  0  0  0  0  0  0  0  0  0  0) Dos_attack(NUMERIC)(1)(0) MITM_attack(NUMERIC)(1)(0) Virus_Attack(NUMERIC)(1)(0) Port_Scan_Attack(NUMERIC)(1)(0) Cyber_Fault(NUMERIC_ARRAY)(10)(0  0  0  0  0  0  0  0  0  0) BGP_hijacking(NUMERIC)(1)(0) Mechanical_Fault(NUMERIC)(1)(0) Conn_Fault(NUMERIC)(1)(0) BotNet_Attack(NUMERIC)(1)(0) Data_Corruption(NUMERIC)(1)(0) SW_Change(NUMERIC)(1)(0) Config_Change(NUMERIC)(1)(0) Port_Saturation(NUMERIC)(1)(0) TLC_revoke(NUMERIC_ARRAY)(20)(0  0  0  0  0  0  0  0  0  0  0  0  0  0  0  0  0  0  0  0)  *** OUTPUT RESOURCES *** NUM_OUTPUTS 4 TLC_CONN (20) TLC_SERVICE (20) CYBER_FAULT (10) SWITCHING_QoS (1), Parameter10=off, codeupdate=off, step_received=Connection=max(Connection_init,TLC_CONN);  TLC_services=max(TLC_services_init,TLC_SERVICE); TLC_services=mod(TLC_services,10); TLC_revoke=floor(TLC_SERVICE/10);  Cyber_Fault=max(CYBER_FAULT, transpose([Dos_attack   MITM_attack Virus_Attack Port_Scan_Attack  BGP_hijacking BotNet_Attack Data_Corruption SW_Change Config_Change Port_Saturation]));  Conn_Fault=max([Dos_attack  Mechanical_Fault  1-POWER 1-ROOM_QoS] );  Operative_Level=(1-Conn_Fault)*max(max(TLC_services),0.5)*(1-0.5*max(Cyber_Fault));, step_computed=, dynamic_computed=, step_sended=TLC_CONN=Connection*(1-Conn_Fault); TLC_SERVICE=TLC_services*(1-Conn_Fault)+10*TLC_revoke;  Cyber_Transmitted=min(Cyber_Fault, transpose([0 0 1 0 1 1 0 0 0 1])); CYBER_FAULT=Cyber_Transmitted*(1-Conn_Fault);   SWITCHING_QoS=Operative_Level;, id_entity=93, id_project=40, id_type=2, name_type=Nexus93180Switch, color=#0072BD}
      mask prompts: Parameter1 "entity name"; Parameter2 "sampling time"; Parameter3 "project"; resources "input resources and state variables"; Parameter10 "Bring state variables to output"; codeupdate "update code from mask"
      mask help: This is a level-2 MATLAB file S-function which demonstrates CISIA entity
      mask DialogControl Container1 Prompt: All parameters
      mask Display: image('Icons/Nexus93180Switch.png')
  OLT_1 (25) : M-S-Function  FunctionName=cisia_msfun  Parameters=Parameter1, Parameter2, Parameter3, resources, Parameter10, codeupdate, step_received, step_computed, dynamic_computed, step_sended, id_entity, id_project, id_type, name_type, color  mask(S-function:msfcn_unit_delay){Parameter1='OLT_1', Parameter2=1, Parameter3='ORO', resources=*** INPUT RESOURCES *** NUM_INPUTS 6 TLC_CONN (20) TLC_SERVICE (20) CYBER_FAULT (10) POWER (1) ROOM_QoS (1) NGPON_IN (20)  *** STATE VARIABLES *** NUM_VARIABLES 22 Operative_Level(NUMERIC)(1)(1) TLC_services(NUMERIC_ARRAY)(20)(0  0  0  0  0  0  0  0  0  0  0  0  0  0  0  0  0  0  0  0) Connection(NUMERIC_ARRAY)(20)(0  0  0  0  0  0  0  0  0  0  0  0  0  0  0  0  0  0  0  0) Dos_attack(NUMERIC)(1)(0) MITM_attack(NUMERIC)(1)(0) Virus_Attack(NUMERIC)(1)(0) Port_Scan_Attack(NUMERIC)(1)(0) Cyber_Fault(NUMERIC_ARRAY)(10)(0  0  0  0  0  0  0  0  0  0) MyConn(NUMERIC_ARRAY)(20)(0  0  0  0  0  0  0  0  0  0  0  0  0  0  0  0  0  0  0  0) BGP_hijacking(NUMERIC)(1)(0) Mechanical_Fault(NUMERIC)(1)(0) Conn_Fault(NUMERIC)(1)(0) Consumed_Services(NUMERIC_ARRAY)(20)(0  0  0  0  0  0  1  0  0  0  0  0  0  0  0  0  0  0  0  0) Service_Fault(NUMERIC)(1)(0) Redundancy_Fault(NUMERIC)(1)(0) BotNet_Attack(NUMERIC)(1)(0) Data_Corruption(NUMERIC)(1)(0) SW_Change(NUMERIC)(1)(0) Config_Change(NUMERIC)(1)(0) Port_Saturation(NUMERIC)(1)(0) My_Service(NUMERIC)(1)(0) TLC_revoke(NUMERIC_ARRAY)(20)(0  0  0  0  0  0  0  0  0  0  0  0  0  0  0  0  0  0  0  0)  *** OUTPUT RESOURCES *** NUM_OUTPUTS 4 TLC_CONN (20) TLC_SERVICE (20) CYBER_FAULT (10) NGPON_CONN (20), Parameter10=off, codeupdate=off, step_received=Connection=max(Connection_init,TLC_CONN); TLC_services=max(TLC_services_init,TLC_SERVICE); TLC_services=mod(TLC_services,10); TLC_revoke=floor(TLC_SERVICE/10);  Cyber_Fault=max(CYBER_FAULT, transpose([Dos_attack   MITM_attack Virus_Attack Port_Scan_Attack  BGP_hijacking BotNet_Attack Data_Corruption SW_Change Config_Change Port_Saturation]));   % Vale 1 in presenza di fault Conn_Fault=max([Dos_attack  Mechanical_Fault  1-POWER 1-ROOM_QoS] );   Service_Fault=max(abs(Consumed_Services.*TLC_services-Consumed_Services));   Redundancy_Fault=max(abs(Consumed_Services.*TLC_CONN-Consumed_Services));  Operative_Level=(1-Conn_Fault)*(1-0.5*max(Cyber_Fault))*(1-Service_Fault)*max(max(TLC_CONN),0.5);   %Operative_Level=(1-Conn_Fault)*max(max(TLC_CONN),0.5)*((2*(1-Service_Fault)+(1-Redundancy_Fault))/3); %My_Service=max([(1-Service_Fault) (1-Redundancy_Fault)/2]); %Operative_Level=(1-Conn_Fault)*My_Service;, step_computed=, dynamic_computed=, step_sended=TLC_CONN=Connection*(1-Conn_Fault); TLC_SERVICE=TLC_services*(1-Conn_Fault)+10*TLC_revoke;  Cyber_Transmitted=min(Cyber_Fault, transpose([0 0 1 0 1 1 0 0 0 1])); CYBER_FAULT=Cyber_Transmitted*(1-Conn_Fault);  NGPON_CONN=TLC_CONN;, id_entity=25, id_project=40, id_type=4, name_type=OLT, color=#FF6929}
      mask prompts: Parameter1 "entity name"; Parameter2 "sampling time"; Parameter3 "project"; resources "input resources and state variables"; Parameter10 "Bring state variables to output"; codeupdate "update code from mask"
      mask help: This is a level-2 MATLAB file S-function which demonstrates CISIA entity
      mask DialogControl Container1 Prompt: All parameters
      mask Display: disp('OLT')
  OLT_2 (57) : M-S-Function  FunctionName=cisia_msfun  Parameters=Parameter1, Parameter2, Parameter3, resources, Parameter10, codeupdate, step_received, step_computed, dynamic_computed, step_sended, id_entity, id_project, id_type, name_type, color  mask(S-function:msfcn_unit_delay){Parameter1='OLT_2', Parameter2=1, Parameter3='ORO', resources=*** INPUT RESOURCES *** NUM_INPUTS 6 TLC_CONN (20) TLC_SERVICE (20) CYBER_FAULT (10) POWER (1) ROOM_QoS (1) NGPON_IN (20)  *** STATE VARIABLES *** NUM_VARIABLES 22 Operative_Level(NUMERIC)(1)(1) TLC_services(NUMERIC_ARRAY)(20)(0  0  0  0  0  0  0  0  0  0  0  0  0  0  0  0  0  0  0  0) Connection(NUMERIC_ARRAY)(20)(0  0  0  0  0  0  0  0  0  0  0  0  0  0  0  0  0  0  0  0) Dos_attack(NUMERIC)(1)(0) MITM_attack(NUMERIC)(1)(0) Virus_Attack(NUMERIC)(1)(0) Port_Scan_Attack(NUMERIC)(1)(0) Cyber_Fault(NUMERIC_ARRAY)(10)(0  0  0  0  0  0  0  0  0  0) MyConn(NUMERIC_ARRAY)(20)(0  0  0  0  0  0  0  0  0  0  0  0  0  0  0  0  0  0  0  0) BGP_hijacking(NUMERIC)(1)(0) Mechanical_Fault(NUMERIC)(1)(0) Conn_Fault(NUMERIC)(1)(0) Consumed_Services(NUMERIC_ARRAY)(20)(0  0  0  0  0  0  1  0  0  0  0  0  0  0  0  0  0  0  0  0) Service_Fault(NUMERIC)(1)(0) Redundancy_Fault(NUMERIC)(1)(0) BotNet_Attack(NUMERIC)(1)(0) Data_Corruption(NUMERIC)(1)(0) SW_Change(NUMERIC)(1)(0) Config_Change(NUMERIC)(1)(0) Port_Saturation(NUMERIC)(1)(0) My_Service(NUMERIC)(1)(0) TLC_revoke(NUMERIC_ARRAY)(20)(0  0  0  0  0  0  0  0  0  0  0  0  0  0  0  0  0  0  0  0)  *** OUTPUT RESOURCES *** NUM_OUTPUTS 4 TLC_CONN (20) TLC_SERVICE (20) CYBER_FAULT (10) NGPON_CONN (20), Parameter10=off, codeupdate=off, step_received=Connection=max(Connection_init,TLC_CONN); TLC_services=max(TLC_services_init,TLC_SERVICE); TLC_services=mod(TLC_services,10); TLC_revoke=floor(TLC_SERVICE/10);  Cyber_Fault=max(CYBER_FAULT, transpose([Dos_attack   MITM_attack Virus_Attack Port_Scan_Attack  BGP_hijacking BotNet_Attack Data_Corruption SW_Change Config_Change Port_Saturation]));   % Vale 1 in presenza di fault Conn_Fault=max([Dos_attack  Mechanical_Fault  1-POWER 1-ROOM_QoS] );   Service_Fault=max(abs(Consumed_Services.*TLC_services-Consumed_Services));   Redundancy_Fault=max(abs(Consumed_Services.*TLC_CONN-Consumed_Services));  Operative_Level=(1-Conn_Fault)*(1-0.5*max(Cyber_Fault))*(1-Service_Fault)*max(max(TLC_CONN),0.5);   %Operative_Level=(1-Conn_Fault)*max(max(TLC_CONN),0.5)*((2*(1-Service_Fault)+(1-Redundancy_Fault))/3); %My_Service=max([(1-Service_Fault) (1-Redundancy_Fault)/2]); %Operative_Level=(1-Conn_Fault)*My_Service;, step_computed=, dynamic_computed=, step_sended=TLC_CONN=Connection*(1-Conn_Fault); TLC_SERVICE=TLC_services*(1-Conn_Fault)+10*TLC_revoke;  Cyber_Transmitted=min(Cyber_Fault, transpose([0 0 1 0 1 1 0 0 0 1])); CYBER_FAULT=Cyber_Transmitted*(1-Conn_Fault);  NGPON_CONN=TLC_CONN;, id_entity=57, id_project=40, id_type=4, name_type=OLT, color=#FF6929}
      mask prompts: Parameter1 "entity name"; Parameter2 "sampling time"; Parameter3 "project"; resources "input resources and state variables"; Parameter10 "Bring state variables to output"; codeupdate "update code from mask"
      mask help: This is a level-2 MATLAB file S-function which demonstrates CISIA entity
      mask DialogControl Container1 Prompt: All parameters
      mask Display: disp('OLT')
  ONU_1 (55) : M-S-Function  FunctionName=cisia_msfun  Parameters=Parameter1, Parameter2, Parameter3, resources, Parameter10, codeupdate, step_received, step_computed, dynamic_computed, step_sended, id_entity, id_project, id_type, name_type, color  mask(S-function:msfcn_unit_delay){Parameter1='ONU_1', Parameter2=1, Parameter3='ORO', resources=*** INPUT RESOURCES *** NUM_INPUTS 4 TLC_SERVICE (20) CYBER_FAULT (10) POWER (1) NGPON_CONN (20)  *** STATE VARIABLES *** NUM_VARIABLES 22 Operative_Level(NUMERIC)(1)(1) TLC_services(NUMERIC_ARRAY)(20)(0  0  0  0  0  0  0  0  0  0  0  0  0  0  0  0  0  0  0  0) Connection(NUMERIC_ARRAY)(20)(0  0  0  0  0  0  0  0  0  0  0  0  0  0  0  0  0  0  0  0) Dos_attack(NUMERIC)(1)(0) MITM_attack(NUMERIC)(1)(0) Virus_Attack(NUMERIC)(1)(0) Port_Scan_Attack(NUMERIC)(1)(0) Cyber_Fault(NUMERIC_ARRAY)(10)(0  0  0  0  0  0  0  0  0  0) MyConn(NUMERIC_ARRAY)(20)(0  0  0  0  0  0  0  0  0  0  0  0  0  0  0  0  0  0  0  0) BGP_hijacking(NUMERIC)(1)(0) Mechanical_Fault(NUMERIC)(1)(0) Conn_Fault(NUMERIC)(1)(0) Consumed_Services(NUMERIC_ARRAY)(20)(0  0  0  0  0  0  0  0  0  0  0  0  0  0  0  0  0  0  0  0) Service_Fault(NUMERIC)(1)(0) Redundancy_Fault(NUMERIC)(1)(0) BotNet_Attack(NUMERIC)(1)(0) Data_Corruption(NUMERIC)(1)(0) SW_Change(NUMERIC)(1)(0) Config_Change(NUMERIC)(1)(0) Port_Saturation(NUMERIC)(1)(0) My_Service(NUMERIC)(1)(0) TLC_revoke(NUMERIC_ARRAY)(20)(0  0  0  0  0  0  0  0  0  0  0  0  0  0  0  0  0  0  0  0)  *** OUTPUT RESOURCES *** NUM_OUTPUTS 3 TLC_SERVICE (20) CYBER_FAULT (10) NGPON_CONN (20), Parameter10=off, codeupdate=off, step_received=Connection=max(Connection_init,NGPON_CONN); TLC_services=max(TLC_services_init,TLC_SERVICE); TLC_services=mod(TLC_services,10); TLC_revoke=floor(TLC_SERVICE/10);  Cyber_Fault=max(CYBER_FAULT, transpose([Dos_attack   MITM_attack Virus_Attack Port_Scan_Attack  BGP_hijacking BotNet_Attack Data_Corruption SW_Change Config_Change Port_Saturation]));  Conn_Fault=max([Dos_attack  Mechanical_Fault  1-POWER] );  Service_Fault=max(abs(Consumed_Services.*TLC_services-Consumed_Services)); Redundancy_Fault=max(abs(Consumed_Services.*NGPON_CONN-Consumed_Services));  Operative_Level=(1-Conn_Fault)*(1-0.5*max(Cyber_Fault))*(1-Service_Fault)*max(max(NGPON_CONN),0.5);  %Operative_Level=(1-Conn_Fault)*max(max(TLC_services),0.5)*((2*(1-Service_Fault)+(1-Redundancy_Fault))/3); % Il servizio utilizzato %My_Service=max([(1-Service_Fault) (1-Redundancy_Fault)/2]); %Operative_Level=(1-Conn_Fault);, step_computed=, dynamic_computed=, step_sended=TLC_SERVICE=TLC_services*(1-Conn_Fault)+10*TLC_revoke; NGPON_CONN=Connection*(1-Conn_Fault);  Cyber_Transmitted=min(Cyber_Fault, transpose([0 0 1 0 1 1 0 0 0 1])); CYBER_FAULT=Cyber_Transmitted*(1-Conn_Fault);, id_entity=55, id_project=40, id_type=12, name_type=ONU, color=#90DB5A}
      mask prompts: Parameter1 "entity name"; Parameter2 "sampling time"; Parameter3 "project"; resources "input resources and state variables"; Parameter10 "Bring state variables to output"; codeupdate "update code from mask"
      mask help: This is a level-2 MATLAB file S-function which demonstrates CISIA entity
      mask DialogControl Container1 Prompt: All parameters
      mask Display: disp('ONU')
  ONU_2 (58) : M-S-Function  FunctionName=cisia_msfun  Parameters=Parameter1, Parameter2, Parameter3, resources, Parameter10, codeupdate, step_received, step_computed, dynamic_computed, step_sended, id_entity, id_project, id_type, name_type, color  mask(S-function:msfcn_unit_delay){Parameter1='ONU_2', Parameter2=1, Parameter3='ORO', resources=*** INPUT RESOURCES *** NUM_INPUTS 4 TLC_SERVICE (20) CYBER_FAULT (10) POWER (1) NGPON_CONN (20)  *** STATE VARIABLES *** NUM_VARIABLES 22 Operative_Level(NUMERIC)(1)(1) TLC_services(NUMERIC_ARRAY)(20)(0  0  0  0  0  0  0  0  0  0  0  0  0  0  0  0  0  0  0  0) Connection(NUMERIC_ARRAY)(20)(0  0  0  0  0  0  0  0  0  0  0  0  0  0  0  0  0  0  0  0) Dos_attack(NUMERIC)(1)(0) MITM_attack(NUMERIC)(1)(0) Virus_Attack(NUMERIC)(1)(0) Port_Scan_Attack(NUMERIC)(1)(0) Cyber_Fault(NUMERIC_ARRAY)(10)(0  0  0  0  0  0  0  0  0  0) MyConn(NUMERIC_ARRAY)(20)(0  0  0  0  0  0  0  0  0  0  0  0  0  0  0  0  0  0  0  0) BGP_hijacking(NUMERIC)(1)(0) Mechanical_Fault(NUMERIC)(1)(0) Conn_Fault(NUMERIC)(1)(0) Consumed_Services(NUMERIC_ARRAY)(20)(0  0  0  0  0  0  0  0  0  0  0  0  0  0  0  0  0  0  0  0) Service_Fault(NUMERIC)(1)(0) Redundancy_Fault(NUMERIC)(1)(0) BotNet_Attack(NUMERIC)(1)(0) Data_Corruption(NUMERIC)(1)(0) SW_Change(NUMERIC)(1)(0) Config_Change(NUMERIC)(1)(0) Port_Saturation(NUMERIC)(1)(0) My_Service(NUMERIC)(1)(0) TLC_revoke(NUMERIC_ARRAY)(20)(0  0  0  0  0  0  0  0  0  0  0  0  0  0  0  0  0  0  0  0)  *** OUTPUT RESOURCES *** NUM_OUTPUTS 3 TLC_SERVICE (20) CYBER_FAULT (10) NGPON_CONN (20), Parameter10=off, codeupdate=off, step_received=Connection=max(Connection_init,NGPON_CONN); TLC_services=max(TLC_services_init,TLC_SERVICE); TLC_services=mod(TLC_services,10); TLC_revoke=floor(TLC_SERVICE/10);  Cyber_Fault=max(CYBER_FAULT, transpose([Dos_attack   MITM_attack Virus_Attack Port_Scan_Attack  BGP_hijacking BotNet_Attack Data_Corruption SW_Change Config_Change Port_Saturation]));  Conn_Fault=max([Dos_attack  Mechanical_Fault  1-POWER] );  Service_Fault=max(abs(Consumed_Services.*TLC_services-Consumed_Services)); Redundancy_Fault=max(abs(Consumed_Services.*NGPON_CONN-Consumed_Services));  Operative_Level=(1-Conn_Fault)*(1-0.5*max(Cyber_Fault))*(1-Service_Fault)*max(max(NGPON_CONN),0.5);  %Operative_Level=(1-Conn_Fault)*max(max(TLC_services),0.5)*((2*(1-Service_Fault)+(1-Redundancy_Fault))/3); % Il servizio utilizzato %My_Service=max([(1-Service_Fault) (1-Redundancy_Fault)/2]); %Operative_Level=(1-Conn_Fault);, step_computed=, dynamic_computed=, step_sended=TLC_SERVICE=TLC_services*(1-Conn_Fault)+10*TLC_revoke; NGPON_CONN=Connection*(1-Conn_Fault);  Cyber_Transmitted=min(Cyber_Fault, transpose([0 0 1 0 1 1 0 0 0 1])); CYBER_FAULT=Cyber_Transmitted*(1-Conn_Fault);, id_entity=58, id_project=40, id_type=12, name_type=ONU, color=#90DB5A}
      mask prompts: Parameter1 "entity name"; Parameter2 "sampling time"; Parameter3 "project"; resources "input resources and state variables"; Parameter10 "Bring state variables to output"; codeupdate "update code from mask"
      mask help: This is a level-2 MATLAB file S-function which demonstrates CISIA entity
      mask DialogControl Container1 Prompt: All parameters
      mask Display: disp('ONU')
  PowerGen_1 (46) : M-S-Function  FunctionName=cisia_msfun  Parameters=Parameter1, Parameter2, Parameter3, resources, Parameter10, codeupdate, step_received, step_computed, dynamic_computed, step_sended, id_entity, id_project, id_type, name_type, color  mask(S-function:msfcn_unit_delay){Parameter1='PowerGen_1', Parameter2=1, Parameter3='ORO', resources=*** INPUT RESOURCES *** NUM_INPUTS 0  *** STATE VARIABLES *** NUM_VARIABLES 2 Operative_Level(NUMERIC)(1)(1) Power_Fault(NUMERIC)(1)(0)  *** OUTPUT RESOURCES *** NUM_OUTPUTS 1 POWER (1), Parameter10=off, codeupdate=off, step_received=Operative_Level=1-Power_Fault;, step_computed=, dynamic_computed=, step_sended=POWER=Operative_Level;, id_entity=46, id_project=40, id_type=8, name_type=PowerSource, color=#84BD8C}
      mask prompts: Parameter1 "entity name"; Parameter2 "sampling time"; Parameter3 "project"; resources "input resources and state variables"; Parameter10 "Bring state variables to output"; codeupdate "update code from mask"
      mask help: This is a level-2 MATLAB file S-function which demonstrates CISIA entity
      mask DialogControl Container1 Prompt: All parameters
      mask Display: image('Icons/PowerSource.png')
  PowerGen_2 (47) : M-S-Function  FunctionName=cisia_msfun  Parameters=Parameter1, Parameter2, Parameter3, resources, Parameter10, codeupdate, step_received, step_computed, dynamic_computed, step_sended, id_entity, id_project, id_type, name_type, color  mask(S-function:msfcn_unit_delay){Parameter1='PowerGen_2', Parameter2=1, Parameter3='ORO', resources=*** INPUT RESOURCES *** NUM_INPUTS 0  *** STATE VARIABLES *** NUM_VARIABLES 2 Operative_Level(NUMERIC)(1)(1) Power_Fault(NUMERIC)(1)(0)  *** OUTPUT RESOURCES *** NUM_OUTPUTS 1 POWER (1), Parameter10=off, codeupdate=off, step_received=Operative_Level=1-Power_Fault;, step_computed=, dynamic_computed=, step_sended=POWER=Operative_Level;, id_entity=47, id_project=40, id_type=8, name_type=PowerSource, color=#84BD8C}
      mask prompts: Parameter1 "entity name"; Parameter2 "sampling time"; Parameter3 "project"; resources "input resources and state variables"; Parameter10 "Bring state variables to output"; codeupdate "update code from mask"
      mask help: This is a level-2 MATLAB file S-function which demonstrates CISIA entity
      mask DialogControl Container1 Prompt: All parameters
      mask Display: image('Icons/PowerSource.png')
  PowerGen_3 (157) : M-S-Function  FunctionName=cisia_msfun  Parameters=Parameter1, Parameter2, Parameter3, resources, Parameter10, codeupdate, step_received, step_computed, dynamic_computed, step_sended, id_entity, id_project, id_type, name_type, color  mask(S-function:msfcn_unit_delay){Parameter1='PowerGen_3', Parameter2=1, Parameter3='ORO', resources=*** INPUT RESOURCES *** NUM_INPUTS 0  *** STATE VARIABLES *** NUM_VARIABLES 2 Operative_Level(NUMERIC)(1)(1) Power_Fault(NUMERIC)(1)(0)  *** OUTPUT RESOURCES *** NUM_OUTPUTS 1 POWER (1), Parameter10=off, codeupdate=off, step_received=Operative_Level=1-Power_Fault;, step_computed=, dynamic_computed=, step_sended=POWER=Operative_Level;, id_entity=157, id_project=40, id_type=8, name_type=PowerSource, color=#84BD8C}
      mask prompts: Parameter1 "entity name"; Parameter2 "sampling time"; Parameter3 "project"; resources "input resources and state variables"; Parameter10 "Bring state variables to output"; codeupdate "update code from mask"
      mask help: This is a level-2 MATLAB file S-function which demonstrates CISIA entity
      mask DialogControl Container1 Prompt: All parameters
      mask Display: image('Icons/PowerSource.png')
  PowerGen_4 (214) : M-S-Function  FunctionName=cisia_msfun  Parameters=Parameter1, Parameter2, Parameter3, resources, Parameter10, codeupdate, step_received, step_computed, dynamic_computed, step_sended, id_entity, id_project, id_type, name_type, color  mask(S-function:msfcn_unit_delay){Parameter1='PowerGen_4', Parameter2=1, Parameter3='ORO', resources=*** INPUT RESOURCES *** NUM_INPUTS 0  *** STATE VARIABLES *** NUM_VARIABLES 2 Operative_Level(NUMERIC)(1)(1) Power_Fault(NUMERIC)(1)(0)  *** OUTPUT RESOURCES *** NUM_OUTPUTS 1 POWER (1), Parameter10=off, codeupdate=off, step_received=Operative_Level=1-Power_Fault;, step_computed=, dynamic_computed=, step_sended=POWER=Operative_Level;, id_entity=214, id_project=40, id_type=8, name_type=PowerSource, color=#84BD8C}
      mask prompts: Parameter1 "entity name"; Parameter2 "sampling time"; Parameter3 "project"; resources "input resources and state variables"; Parameter10 "Bring state variables to output"; codeupdate "update code from mask"
      mask help: This is a level-2 MATLAB file S-function which demonstrates CISIA entity
      mask DialogControl Container1 Prompt: All parameters
      mask Display: image('Icons/PowerSource.png')
  PowerGen_5 (236) : M-S-Function  FunctionName=cisia_msfun  Parameters=Parameter1, Parameter2, Parameter3, resources, Parameter10, codeupdate, step_received, step_computed, dynamic_computed, step_sended, id_entity, id_project, id_type, name_type, color  mask(S-function:msfcn_unit_delay){Parameter1='PowerGen_5', Parameter2=1, Parameter3='ORO', resources=*** INPUT RESOURCES *** NUM_INPUTS 0  *** STATE VARIABLES *** NUM_VARIABLES 2 Operative_Level(NUMERIC)(1)(1) Power_Fault(NUMERIC)(1)(0)  *** OUTPUT RESOURCES *** NUM_OUTPUTS 1 POWER (1), Parameter10=off, codeupdate=off, step_received=Operative_Level=1-Power_Fault;, step_computed=, dynamic_computed=, step_sended=POWER=Operative_Level;, id_entity=236, id_project=40, id_type=8, name_type=PowerSource, color=#84BD8C}
      mask prompts: Parameter1 "entity name"; Parameter2 "sampling time"; Parameter3 "project"; resources "input resources and state variables"; Parameter10 "Bring state variables to output"; codeupdate "update code from mask"
      mask help: This is a level-2 MATLAB file S-function which demonstrates CISIA entity
      mask DialogControl Container1 Prompt: All parameters
      mask Display: image('Icons/PowerSource.png')
  ROOM_1 (51) : M-S-Function  FunctionName=cisia_msfun  Parameters=Parameter1, Parameter2, Parameter3, resources, Parameter10, codeupdate, step_received, step_computed, dynamic_computed, step_sended, id_entity, id_project, id_type, name_type, color  mask(S-function:msfcn_unit_delay){Parameter1='ROOM_1', Parameter2=1, Parameter3='ORO', resources=*** INPUT RESOURCES *** NUM_INPUTS 1 POWER (1)  *** STATE VARIABLES *** NUM_VARIABLES 8 Operative_Level(NUMERIC)(1)(1) Power_Fault(NUMERIC)(1)(0) Cooling_Fault(NUMERIC)(1)(0) Flooding_Fault(NUMERIC)(1)(0) Fire_Fault(NUMERIC)(1)(0) Unauthorized_Access(NUMERIC)(1)(0) Earthquake_Fault(NUMERIC)(1)(0) Physical_Fault(NUMERIC)(1)(0)  *** OUTPUT RESOURCES *** NUM_OUTPUTS 1 ROOM_QoS (1), Parameter10=off, codeupdate=off, step_received=Physical_Fault=max([Power_Fault Flooding_Fault Fire_Fault Cooling_Fault 1-POWER]);   %Operative_Level=min([1-Power_Fault 1-Flooding_Fault  1-Fire_Fault  1-Cooling_Fault  POWER]); %Operative_Level=Operative_Level*max((1-Unauthorized_Access),0.5);  Operative_Level=(1-Physical_Fault)*(1-0.5*Unauthorized_Access);, step_computed=, dynamic_computed=, step_sended=ROOM_QoS=Operative_Level;, id_entity=51, id_project=40, id_type=9, name_type=Room, color=#EDB120}
      mask prompts: Parameter1 "entity name"; Parameter2 "sampling time"; Parameter3 "project"; resources "input resources and state variables"; Parameter10 "Bring state variables to output"; codeupdate "update code from mask"
      mask help: This is a level-2 MATLAB file S-function which demonstrates CISIA entity
      mask DialogControl Container1 Prompt: All parameters
      mask Display: image('Icons/Room.png')
  ROOM_2 (52) : M-S-Function  FunctionName=cisia_msfun  Parameters=Parameter1, Parameter2, Parameter3, resources, Parameter10, codeupdate, step_received, step_computed, dynamic_computed, step_sended, id_entity, id_project, id_type, name_type, color  mask(S-function:msfcn_unit_delay){Parameter1='ROOM_2', Parameter2=1, Parameter3='ORO', resources=*** INPUT RESOURCES *** NUM_INPUTS 1 POWER (1)  *** STATE VARIABLES *** NUM_VARIABLES 8 Operative_Level(NUMERIC)(1)(1) Power_Fault(NUMERIC)(1)(0) Cooling_Fault(NUMERIC)(1)(0) Flooding_Fault(NUMERIC)(1)(0) Fire_Fault(NUMERIC)(1)(0) Unauthorized_Access(NUMERIC)(1)(0) Earthquake_Fault(NUMERIC)(1)(0) Physical_Fault(NUMERIC)(1)(0)  *** OUTPUT RESOURCES *** NUM_OUTPUTS 1 ROOM_QoS (1), Parameter10=off, codeupdate=off, step_received=Physical_Fault=max([Power_Fault Flooding_Fault Fire_Fault Cooling_Fault 1-POWER]);   %Operative_Level=min([1-Power_Fault 1-Flooding_Fault  1-Fire_Fault  1-Cooling_Fault  POWER]); %Operative_Level=Operative_Level*max((1-Unauthorized_Access),0.5);  Operative_Level=(1-Physical_Fault)*(1-0.5*Unauthorized_Access);, step_computed=, dynamic_computed=, step_sended=ROOM_QoS=Operative_Level;, id_entity=52, id_project=40, id_type=9, name_type=Room, color=#EDB120}
      mask prompts: Parameter1 "entity name"; Parameter2 "sampling time"; Parameter3 "project"; resources "input resources and state variables"; Parameter10 "Bring state variables to output"; codeupdate "update code from mask"
      mask help: This is a level-2 MATLAB file S-function which demonstrates CISIA entity
      mask DialogControl Container1 Prompt: All parameters
      mask Display: image('Icons/Room.png')
  ROUTE_AL_2 (4) : M-S-Function  FunctionName=cisia_msfun  Parameters=Parameter1, Parameter2, Parameter3, Parameter4, Parameter5, Parameter6, Parameter7  mask(S-function:msfcn_unit_delay){Parameter1='ROUTE_AL_2', Parameter2=1, Parameter3='ORO', Parameter4=4, Parameter5=0, Parameter6=20, Parameter7=off}
      mask prompts: Parameter1 "entity name"; Parameter2 "sampling time"; Parameter3 "project"; Parameter4 "number of output links"; Parameter5 "default value for outputs"; Parameter6 "link dimension (unused))"; Parameter7 "select resource elements and output port from input"
      mask help: This is a level-2 MATLAB file S-function which demonstrates CISIA entity
      mask Display: disp('ROUTE')
  ROUTE_AL_3 (5) : M-S-Function  FunctionName=cisia_msfun  Parameters=Parameter1, Parameter2, Parameter3, Parameter4, Parameter5, Parameter6, Parameter7  mask(S-function:msfcn_unit_delay){Parameter1='ROUTE_AL_3', Parameter2=1, Parameter3='ORO', Parameter4=2, Parameter5=0, Parameter6=20, Parameter7=off}
      mask prompts: Parameter1 "entity name"; Parameter2 "sampling time"; Parameter3 "project"; Parameter4 "number of output links"; Parameter5 "default value for outputs"; Parameter6 "link dimension (unused))"; Parameter7 "select resource elements and output port from input"
      mask help: This is a level-2 MATLAB file S-function which demonstrates CISIA entity
      mask Display: disp('ROUTE')
  ROUTE_AL_4 (6) : M-S-Function  FunctionName=cisia_msfun  Parameters=Parameter1, Parameter2, Parameter3, Parameter4, Parameter5, Parameter6, Parameter7  mask(S-function:msfcn_unit_delay){Parameter1='ROUTE_AL_4', Parameter2=1, Parameter3='ORO', Parameter4=2, Parameter5=0, Parameter6=20, Parameter7=off}
      mask prompts: Parameter1 "entity name"; Parameter2 "sampling time"; Parameter3 "project"; Parameter4 "number of output links"; Parameter5 "default value for outputs"; Parameter6 "link dimension (unused))"; Parameter7 "select resource elements and output port from input"
      mask help: This is a level-2 MATLAB file S-function which demonstrates CISIA entity
      mask Display: disp('ROUTE')
  R_Wire_1 (98) : M-S-Function  FunctionName=cisia_msfun  Parameters=Parameter1, Parameter2, Parameter3, resources, Parameter10, codeupdate, step_received, step_computed, dynamic_computed, step_sended, id_entity, id_project, id_type, name_type, color  mask(S-function:msfcn_unit_delay){Parameter1='R_Wire_1', Parameter2=1, Parameter3='ORO', resources=*** INPUT RESOURCES *** NUM_INPUTS 4 TLC_CONN (20) TLC_SERVICE (20) CYBER_FAULT (10) MECH_FAULT (1)  *** STATE VARIABLES *** NUM_VARIABLES 8 Operative_Level(NUMERIC)(1)(1) TLC_services(NUMERIC_ARRAY)(20)(0  0  0  0  0  0  0  0  0  0  0  0  0  0  0  0  0  0  0  0) Connection(NUMERIC_ARRAY)(20)(0  0  0  0  0  0  0  0  0  0  0  0  0  0  0  0  0  0  0  0) Dos_attack(NUMERIC)(1)(0) Cyber_Fault(NUMERIC_ARRAY)(10)(0  0  0  0  0  0  0  0  0  0) Mechanical_Fault(NUMERIC)(1)(0) Conn_Fault(NUMERIC)(1)(0) TLC_revoke(NUMERIC_ARRAY)(20)(0  0  0  0  0  0  0  0  0  0  0  0  0  0  0  0  0  0  0  0)  *** OUTPUT RESOURCES *** NUM_OUTPUTS 4 TLC_CONN (20) TLC_SERVICE (20) CYBER_FAULT (10) MECH_FAULT (1), Parameter10=off, codeupdate=off, step_received=Connection=max(Connection_init,TLC_CONN); TLC_services=max(TLC_services_init,TLC_SERVICE); TLC_services=mod(TLC_services,10); TLC_revoke=floor(TLC_SERVICE/10);  Cyber_Fault=CYBER_FAULT;  Mechanical_Fault=max([Mechanical_Fault MECH_FAULT Mechanical_Fault_init]);  %TLC_services=TLC_services.*(1-TLC_revoke);  Operative_Level=1-Mechanical_Fault;, step_computed=, dynamic_computed=, step_sended=TLC_CONN=Connection*Operative_Level; TLC_SERVICE=TLC_services*Operative_Level+10*TLC_revoke; CYBER_FAULT=Cyber_Fault*Operative_Level; MECH_FAULT=Mechanical_Fault;, id_entity=98, id_project=40, id_type=21, name_type=Redundant_Wire, color=#038F03}
      mask prompts: Parameter1 "entity name"; Parameter2 "sampling time"; Parameter3 "project"; resources "input resources and state variables"; Parameter10 "Bring state variables to output"; codeupdate "update code from mask"
      mask help: This is a level-2 MATLAB file S-function which demonstrates CISIA entity
      mask DialogControl Container1 Prompt: All parameters
      mask Display: disp('Redundant_Wire')
  R_Wire_1b (99) : M-S-Function  FunctionName=cisia_msfun  Parameters=Parameter1, Parameter2, Parameter3, resources, Parameter10, codeupdate, step_received, step_computed, dynamic_computed, step_sended, id_entity, id_project, id_type, name_type, color  mask(S-function:msfcn_unit_delay){Parameter1='R_Wire_1b', Parameter2=1, Parameter3='ORO', resources=*** INPUT RESOURCES *** NUM_INPUTS 4 TLC_CONN (20) TLC_SERVICE (20) CYBER_FAULT (10) MECH_FAULT (1)  *** STATE VARIABLES *** NUM_VARIABLES 8 Operative_Level(NUMERIC)(1)(1) TLC_services(NUMERIC_ARRAY)(20)(0  0  0  0  0  0  0  0  0  0  0  0  0  0  0  0  0  0  0  0) Connection(NUMERIC_ARRAY)(20)(0  0  0  0  0  0  0  0  0  0  0  0  0  0  0  0  0  0  0  0) Dos_attack(NUMERIC)(1)(0) Cyber_Fault(NUMERIC_ARRAY)(10)(0  0  0  0  0  0  0  0  0  0) Mechanical_Fault(NUMERIC)(1)(0) Conn_Fault(NUMERIC)(1)(0) TLC_revoke(NUMERIC_ARRAY)(20)(0  0  0  0  0  0  0  0  0  0  0  0  0  0  0  0  0  0  0  0)  *** OUTPUT RESOURCES *** NUM_OUTPUTS 4 TLC_CONN (20) TLC_SERVICE (20) CYBER_FAULT (10) MECH_FAULT (1), Parameter10=off, codeupdate=off, step_received=Connection=max(Connection_init,TLC_CONN); TLC_services=max(TLC_services_init,TLC_SERVICE); TLC_services=mod(TLC_services,10); TLC_revoke=floor(TLC_SERVICE/10);  Cyber_Fault=CYBER_FAULT;  Mechanical_Fault=max([Mechanical_Fault MECH_FAULT Mechanical_Fault_init]);  %TLC_services=TLC_services.*(1-TLC_revoke);  Operative_Level=1-Mechanical_Fault;, step_computed=, dynamic_computed=, step_sended=TLC_CONN=Connection*Operative_Level; TLC_SERVICE=TLC_services*Operative_Level+10*TLC_revoke; CYBER_FAULT=Cyber_Fault*Operative_Level; MECH_FAULT=Mechanical_Fault;, id_entity=99, id_project=40, id_type=21, name_type=Redundant_Wire, color=#038F03}
      mask prompts: Parameter1 "entity name"; Parameter2 "sampling time"; Parameter3 "project"; resources "input resources and state variables"; Parameter10 "Bring state variables to output"; codeupdate "update code from mask"
      mask help: This is a level-2 MATLAB file S-function which demonstrates CISIA entity
      mask DialogControl Container1 Prompt: All parameters
      mask Display: disp('Redundant_Wire')
  Redundancy : Constant
  Room_6 (241) : M-S-Function  FunctionName=cisia_msfun  Parameters=Parameter1, Parameter2, Parameter3, resources, Parameter10, codeupdate, step_received, step_computed, dynamic_computed, step_sended, id_entity, id_project, id_type, name_type, color  mask(S-function:msfcn_unit_delay){Parameter1='Room_6', Parameter2=1, Parameter3='ORO', resources=*** INPUT RESOURCES *** NUM_INPUTS 1 POWER (1)  *** STATE VARIABLES *** NUM_VARIABLES 8 Operative_Level(NUMERIC)(1)(1) Power_Fault(NUMERIC)(1)(0) Cooling_Fault(NUMERIC)(1)(0) Flooding_Fault(NUMERIC)(1)(0) Fire_Fault(NUMERIC)(1)(0) Unauthorized_Access(NUMERIC)(1)(0) Earthquake_Fault(NUMERIC)(1)(0) Physical_Fault(NUMERIC)(1)(0)  *** OUTPUT RESOURCES *** NUM_OUTPUTS 1 ROOM_QoS (1), Parameter10=off, codeupdate=off, step_received=Physical_Fault=max([Power_Fault Flooding_Fault Fire_Fault Cooling_Fault 1-POWER]);   %Operative_Level=min([1-Power_Fault 1-Flooding_Fault  1-Fire_Fault  1-Cooling_Fault  POWER]); %Operative_Level=Operative_Level*max((1-Unauthorized_Access),0.5);  Operative_Level=(1-Physical_Fault)*(1-0.5*Unauthorized_Access);, step_computed=, dynamic_computed=, step_sended=ROOM_QoS=Operative_Level;, id_entity=241, id_project=40, id_type=9, name_type=Room, color=#EDB120}
      mask prompts: Parameter1 "entity name"; Parameter2 "sampling time"; Parameter3 "project"; resources "input resources and state variables"; Parameter10 "Bring state variables to output"; codeupdate "update code from mask"
      mask help: This is a level-2 MATLAB file S-function which demonstrates CISIA entity
      mask DialogControl Container1 Prompt: All parameters
      mask Display: image('Icons/Room.png')
  SAVE_1 (1) : M-S-Function  FunctionName=cisia_msfun  Parameters=Parameter1, Parameter2, Parameter3, Parameter4,Parameter5,Parameter6,Parameter7  mask(S-function:msfcn_unit_delay){Parameter1='SAVE_1', Parameter2=1, Parameter3='SistemiIoT', Parameter4=on, Parameter5=[1], Parameter6=[1], Parameter7=off}
      mask prompts: Parameter1 "entity name"; Parameter2 "sampling time"; Parameter3 "project"; Parameter4 "display bars"; Parameter5 "values"; Parameter6 "logic"; Parameter7 "display B/W"
      mask help: This is a level-2 MATLAB file S-function which demonstrates CISIA entity
      mask DialogControl Container3 Prompt: Display
      mask Display: disp('SAVE')
  SAVE_11 (11) : M-S-Function  FunctionName=cisia_msfun  Parameters=Parameter1, Parameter2, Parameter3, Parameter4,Parameter5,Parameter6,Parameter7  mask(S-function:msfcn_unit_delay){Parameter1='SAVE_11', Parameter2=1, Parameter3='SistemiIoT', Parameter4=on, Parameter5=[1], Parameter6=[1], Parameter7=off}
      mask prompts: Parameter1 "entity name"; Parameter2 "sampling time"; Parameter3 "project"; Parameter4 "display bars"; Parameter5 "values"; Parameter6 "logic"; Parameter7 "display B/W"
      mask help: This is a level-2 MATLAB file S-function which demonstrates CISIA entity
      mask DialogControl Container3 Prompt: Display
      mask Display: disp('SAVE')
  SAVE_2 (2) : M-S-Function  FunctionName=cisia_msfun  Parameters=Parameter1, Parameter2, Parameter3, Parameter4,Parameter5,Parameter6,Parameter7  mask(S-function:msfcn_unit_delay){Parameter1='SAVE_2', Parameter2=1, Parameter3='SistemiIoT', Parameter4=on, Parameter5=[1], Parameter6=[1], Parameter7=off}
      mask prompts: Parameter1 "entity name"; Parameter2 "sampling time"; Parameter3 "project"; Parameter4 "display bars"; Parameter5 "values"; Parameter6 "logic"; Parameter7 "display B/W"
      mask help: This is a level-2 MATLAB file S-function which demonstrates CISIA entity
      mask DialogControl Container3 Prompt: Display
      mask Display: disp('SAVE')
  SAVE_20 (20) : M-S-Function  FunctionName=cisia_msfun  Parameters=Parameter1, Parameter2, Parameter3, Parameter4,Parameter5,Parameter6,Parameter7  mask(S-function:msfcn_unit_delay){Parameter1='SAVE_20', Parameter2=1, Parameter3='SistemiIoT', Parameter4=on, Parameter5=[1], Parameter6=[1], Parameter7=off}
      mask prompts: Parameter1 "entity name"; Parameter2 "sampling time"; Parameter3 "project"; Parameter4 "display bars"; Parameter5 "values"; Parameter6 "logic"; Parameter7 "display B/W"
      mask help: This is a level-2 MATLAB file S-function which demonstrates CISIA entity
      mask DialogControl Container3 Prompt: Display
      mask Display: disp('SAVE')
  SAVE_21 (21) : M-S-Function  FunctionName=cisia_msfun  Parameters=Parameter1, Parameter2, Parameter3, Parameter4,Parameter5,Parameter6,Parameter7  mask(S-function:msfcn_unit_delay){Parameter1='SAVE_21', Parameter2=1, Parameter3='ORO', Parameter4=on, Parameter5=[0], Parameter6=[1], Parameter7=off}
      mask prompts: Parameter1 "entity name"; Parameter2 "sampling time"; Parameter3 "project"; Parameter4 "display bars"; Parameter5 "values"; Parameter6 "logic"; Parameter7 "display B/W"
      mask help: This is a level-2 MATLAB file S-function which demonstrates CISIA entity
      mask DialogControl Container3 Prompt: Display
      mask Display: disp('SAVE')
  SAVE_22 (22) : M-S-Function  FunctionName=cisia_msfun  Parameters=Parameter1, Parameter2, Parameter3, Parameter4,Parameter5,Parameter6,Parameter7  mask(S-function:msfcn_unit_delay){Parameter1='SAVE_22', Parameter2=1, Parameter3='SistemiIoT', Parameter4=on, Parameter5=[1], Parameter6=[1], Parameter7=off}
      mask prompts: Parameter1 "entity name"; Parameter2 "sampling time"; Parameter3 "project"; Parameter4 "display bars"; Parameter5 "values"; Parameter6 "logic"; Parameter7 "display B/W"
      mask help: This is a level-2 MATLAB file S-function which demonstrates CISIA entity
      mask DialogControl Container3 Prompt: Display
      mask Display: disp('SAVE')
  SAVE_3 (3) : M-S-Function  FunctionName=cisia_msfun  Parameters=Parameter1, Parameter2, Parameter3, Parameter4,Parameter5,Parameter6,Parameter7  mask(S-function:msfcn_unit_delay){Parameter1='SAVE_3', Parameter2=1, Parameter3='SistemiIoT', Parameter4=on, Parameter5=[1], Parameter6=[1], Parameter7=off}
      mask prompts: Parameter1 "entity name"; Parameter2 "sampling time"; Parameter3 "project"; Parameter4 "display bars"; Parameter5 "values"; Parameter6 "logic"; Parameter7 "display B/W"
      mask help: This is a level-2 MATLAB file S-function which demonstrates CISIA entity
      mask DialogControl Container3 Prompt: Display
      mask Display: disp('SAVE')
  SAVE_4 (4) : M-S-Function  FunctionName=cisia_msfun  Parameters=Parameter1, Parameter2, Parameter3, Parameter4,Parameter5,Parameter6,Parameter7  mask(S-function:msfcn_unit_delay){Parameter1='SAVE_4', Parameter2=1, Parameter3='SistemiIoT', Parameter4=on, Parameter5=[1], Parameter6=[1], Parameter7=off}
      mask prompts: Parameter1 "entity name"; Parameter2 "sampling time"; Parameter3 "project"; Parameter4 "display bars"; Parameter5 "values"; Parameter6 "logic"; Parameter7 "display B/W"
      mask help: This is a level-2 MATLAB file S-function which demonstrates CISIA entity
      mask DialogControl Container3 Prompt: Display
      mask Display: disp('SAVE')
  SAVE_5 (5) : M-S-Function  FunctionName=cisia_msfun  Parameters=Parameter1, Parameter2, Parameter3, Parameter4,Parameter5,Parameter6,Parameter7  mask(S-function:msfcn_unit_delay){Parameter1='SAVE_5', Parameter2=1, Parameter3='SistemiIoT', Parameter4=on, Parameter5=[1], Parameter6=[1], Parameter7=off}
      mask prompts: Parameter1 "entity name"; Parameter2 "sampling time"; Parameter3 "project"; Parameter4 "display bars"; Parameter5 "values"; Parameter6 "logic"; Parameter7 "display B/W"
      mask help: This is a level-2 MATLAB file S-function which demonstrates CISIA entity
      mask DialogControl Container3 Prompt: Display
      mask Display: disp('SAVE')
  SAVE_6 (6) : M-S-Function  FunctionName=cisia_msfun  Parameters=Parameter1, Parameter2, Parameter3, Parameter4,Parameter5,Parameter6,Parameter7  mask(S-function:msfcn_unit_delay){Parameter1='SAVE_6', Parameter2=1, Parameter3='SistemiIoT', Parameter4=on, Parameter5=[1], Parameter6=[1], Parameter7=off}
      mask prompts: Parameter1 "entity name"; Parameter2 "sampling time"; Parameter3 "project"; Parameter4 "display bars"; Parameter5 "values"; Parameter6 "logic"; Parameter7 "display B/W"
      mask help: This is a level-2 MATLAB file S-function which demonstrates CISIA entity
      mask DialogControl Container3 Prompt: Display
      mask Display: disp('SAVE')
  SAVE_7 (7) : M-S-Function  FunctionName=cisia_msfun  Parameters=Parameter1, Parameter2, Parameter3, Parameter4,Parameter5,Parameter6,Parameter7  mask(S-function:msfcn_unit_delay){Parameter1='SAVE_7', Parameter2=1, Parameter3='SistemiIoT', Parameter4=on, Parameter5=[1], Parameter6=[1], Parameter7=off}
      mask prompts: Parameter1 "entity name"; Parameter2 "sampling time"; Parameter3 "project"; Parameter4 "display bars"; Parameter5 "values"; Parameter6 "logic"; Parameter7 "display B/W"
      mask help: This is a level-2 MATLAB file S-function which demonstrates CISIA entity
      mask DialogControl Container3 Prompt: Display
      mask Display: disp('SAVE')
  SAVE_8 (8) : M-S-Function  FunctionName=cisia_msfun  Parameters=Parameter1, Parameter2, Parameter3, Parameter4,Parameter5,Parameter6,Parameter7  mask(S-function:msfcn_unit_delay){Parameter1='SAVE_8', Parameter2=1, Parameter3='SistemiIoT', Parameter4=on, Parameter5=[1], Parameter6=[1], Parameter7=off}
      mask prompts: Parameter1 "entity name"; Parameter2 "sampling time"; Parameter3 "project"; Parameter4 "display bars"; Parameter5 "values"; Parameter6 "logic"; Parameter7 "display B/W"
      mask help: This is a level-2 MATLAB file S-function which demonstrates CISIA entity
      mask DialogControl Container3 Prompt: Display
      mask Display: disp('SAVE')
  SAVE_9 (9) : M-S-Function  FunctionName=cisia_msfun  Parameters=Parameter1, Parameter2, Parameter3, Parameter4,Parameter5,Parameter6,Parameter7  mask(S-function:msfcn_unit_delay){Parameter1='SAVE_9', Parameter2=1, Parameter3='SistemiIoT', Parameter4=on, Parameter5=[1], Parameter6=[1], Parameter7=off}
      mask prompts: Parameter1 "entity name"; Parameter2 "sampling time"; Parameter3 "project"; Parameter4 "display bars"; Parameter5 "values"; Parameter6 "logic"; Parameter7 "display B/W"
      mask help: This is a level-2 MATLAB file S-function which demonstrates CISIA entity
      mask DialogControl Container3 Prompt: Display
      mask Display: disp('SAVE')
  Splitter_1 (54) : M-S-Function  FunctionName=cisia_msfun  Parameters=Parameter1, Parameter2, Parameter3, resources, Parameter10, codeupdate, step_received, step_computed, dynamic_computed, step_sended, id_entity, id_project, id_type, name_type, color  mask(S-function:msfcn_unit_delay){Parameter1='Splitter_1', Parameter2=1, Parameter3='ORO', resources=*** INPUT RESOURCES *** NUM_INPUTS 3 TLC_SERVICE (20) CYBER_FAULT (10) NGPON_CONN (20)  *** STATE VARIABLES *** NUM_VARIABLES 18 Operative_Level(NUMERIC)(1)(1) TLC_services(NUMERIC_ARRAY)(20)(0  0  0  0  0  0  0  0  0  0  0  0  0  0  0  0  0  0  0  0) Connection(NUMERIC_ARRAY)(20)(0  0  0  0  0  0  0  0  0  0  0  0  0  0  0  0  0  0  0  0) Dos_attack(NUMERIC)(1)(0) MITM_attack(NUMERIC)(1)(0) Virus_Attack(NUMERIC)(1)(0) Port_Scan_Attack(NUMERIC)(1)(0) Cyber_Fault(NUMERIC_ARRAY)(10)(0  0  0  0  0  0  0  0  0  0) MyConn(NUMERIC_ARRAY)(20)(0  0  0  0  0  0  0  0  0  0  0  0  0  0  0  0  0  0  0  0) BGP_hijacking(NUMERIC)(1)(0) Mechanical_Fault(NUMERIC)(1)(0) Conn_Fault(NUMERIC)(1)(0) BotNet_Attack(NUMERIC)(1)(0) Data_Corruption(NUMERIC)(1)(0) SW_Change(NUMERIC)(1)(0) Config_Change(NUMERIC)(1)(0) Port_Saturation(NUMERIC)(1)(0) TLC_revoke(NUMERIC_ARRAY)(20)(0  0  0  0  0  0  0  0  0  0  0  0  0  0  0  0  0  0  0  0)  *** OUTPUT RESOURCES *** NUM_OUTPUTS 4 TLC_SERVICE (20) CYBER_FAULT (10) NGPON_CONN (20) NGPON_IN (20), Parameter10=off, codeupdate=off, step_received=Connection=max(Connection_init,NGPON_CONN); TLC_services=max(TLC_services_init,TLC_SERVICE); TLC_services=mod(TLC_services,10); TLC_revoke=floor(TLC_SERVICE/10);  Cyber_Fault=max(CYBER_FAULT, transpose([Dos_attack   MITM_attack Virus_Attack Port_Scan_Attack  BGP_hijacking BotNet_Attack Data_Corruption SW_Change Config_Change Port_Saturation]));  % Vale 1 in presenza di fault Conn_Fault=max([Dos_attack  Mechanical_Fault] );  Operative_Level=(1-Conn_Fault)*max(max(NGPON_CONN),0.5)*(1-0.5*max(Cyber_Fault)) ;, step_computed=, dynamic_computed=, step_sended=NGPON_IN=Connection;  NGPON_CONN=Connection*(1-Conn_Fault); TLC_SERVICE=TLC_services*(1-Conn_Fault)+10*TLC_revoke;  Cyber_Transmitted=min(Cyber_Fault, transpose([0 0 1 0 1 1 0 0 0 1])); CYBER_FAULT=Cyber_Transmitted*(1-Conn_Fault);   ROUTING_QoS=Operative_Level;, id_entity=54, id_project=40, id_type=11, name_type=Splitter, color=#90DB5A}
      mask prompts: Parameter1 "entity name"; Parameter2 "sampling time"; Parameter3 "project"; resources "input resources and state variables"; Parameter10 "Bring state variables to output"; codeupdate "update code from mask"
      mask help: This is a level-2 MATLAB file S-function which demonstrates CISIA entity
      mask DialogControl Container1 Prompt: All parameters
      mask Display: disp('Splitter')
  Splitter_2 (59) : M-S-Function  FunctionName=cisia_msfun  Parameters=Parameter1, Parameter2, Parameter3, resources, Parameter10, codeupdate, step_received, step_computed, dynamic_computed, step_sended, id_entity, id_project, id_type, name_type, color  mask(S-function:msfcn_unit_delay){Parameter1='Splitter_2', Parameter2=1, Parameter3='ORO', resources=*** INPUT RESOURCES *** NUM_INPUTS 3 TLC_SERVICE (20) CYBER_FAULT (10) NGPON_CONN (20)  *** STATE VARIABLES *** NUM_VARIABLES 18 Operative_Level(NUMERIC)(1)(1) TLC_services(NUMERIC_ARRAY)(20)(0  0  0  0  0  0  0  0  0  0  0  0  0  0  0  0  0  0  0  0) Connection(NUMERIC_ARRAY)(20)(0  0  0  0  0  0  0  0  0  0  0  0  0  0  0  0  0  0  0  0) Dos_attack(NUMERIC)(1)(0) MITM_attack(NUMERIC)(1)(0) Virus_Attack(NUMERIC)(1)(0) Port_Scan_Attack(NUMERIC)(1)(0) Cyber_Fault(NUMERIC_ARRAY)(10)(0  0  0  0  0  0  0  0  0  0) MyConn(NUMERIC_ARRAY)(20)(0  0  0  0  0  0  0  0  0  0  0  0  0  0  0  0  0  0  0  0) BGP_hijacking(NUMERIC)(1)(0) Mechanical_Fault(NUMERIC)(1)(0) Conn_Fault(NUMERIC)(1)(0) BotNet_Attack(NUMERIC)(1)(0) Data_Corruption(NUMERIC)(1)(0) SW_Change(NUMERIC)(1)(0) Config_Change(NUMERIC)(1)(0) Port_Saturation(NUMERIC)(1)(0) TLC_revoke(NUMERIC_ARRAY)(20)(0  0  0  0  0  0  0  0  0  0  0  0  0  0  0  0  0  0  0  0)  *** OUTPUT RESOURCES *** NUM_OUTPUTS 4 TLC_SERVICE (20) CYBER_FAULT (10) NGPON_CONN (20) NGPON_IN (20), Parameter10=off, codeupdate=off, step_received=Connection=max(Connection_init,NGPON_CONN); TLC_services=max(TLC_services_init,TLC_SERVICE); TLC_services=mod(TLC_services,10); TLC_revoke=floor(TLC_SERVICE/10);  Cyber_Fault=max(CYBER_FAULT, transpose([Dos_attack   MITM_attack Virus_Attack Port_Scan_Attack  BGP_hijacking BotNet_Attack Data_Corruption SW_Change Config_Change Port_Saturation]));  % Vale 1 in presenza di fault Conn_Fault=max([Dos_attack  Mechanical_Fault] );  Operative_Level=(1-Conn_Fault)*max(max(NGPON_CONN),0.5)*(1-0.5*max(Cyber_Fault)) ;, step_computed=, dynamic_computed=, step_sended=NGPON_IN=Connection;  NGPON_CONN=Connection*(1-Conn_Fault); TLC_SERVICE=TLC_services*(1-Conn_Fault)+10*TLC_revoke;  Cyber_Transmitted=min(Cyber_Fault, transpose([0 0 1 0 1 1 0 0 0 1])); CYBER_FAULT=Cyber_Transmitted*(1-Conn_Fault);   ROUTING_QoS=Operative_Level;, id_entity=59, id_project=40, id_type=11, name_type=Splitter, color=#90DB5A}
      mask prompts: Parameter1 "entity name"; Parameter2 "sampling time"; Parameter3 "project"; resources "input resources and state variables"; Parameter10 "Bring state variables to output"; codeupdate "update code from mask"
      mask help: This is a level-2 MATLAB file S-function which demonstrates CISIA entity
      mask DialogControl Container1 Prompt: All parameters
      mask Display: disp('Splitter')
  Subsystem : Subsystem
  Subsystem10 : Subsystem
  Subsystem5 : Subsystem
  Subsystem7 : Subsystem
  Subsystem8 : Subsystem
  TLC_conn1 : MinMax  Function=max  Inputs=4
  TLC_conn2 : MinMax  Function=max  Inputs=4
  TLC_conn{3..5,9} (4 alike) : MinMax  Function=max  Inputs=2
  TLC_service1 : MinMax  Function=max  Inputs=4
  TLC_service2 : MinMax  Function=max  Inputs=4
  TLC_service{3..5,9} (4 alike) : MinMax  Function=max  Inputs=2
  Wire_10 (30) : M-S-Function  FunctionName=cisia_msfun  Parameters=Parameter1, Parameter2, Parameter3, resources, Parameter10, codeupdate, step_received, step_computed, dynamic_computed, step_sended, id_entity, id_project, id_type, name_type, color  mask(S-function:msfcn_unit_delay){Parameter1='Wire_10', Parameter2=1, Parameter3='ORO', resources=*** INPUT RESOURCES *** NUM_INPUTS 4 TLC_CONN (20) TLC_SERVICE (20) CYBER_FAULT (10) MECH_FAULT (1)  *** STATE VARIABLES *** NUM_VARIABLES 11 Operative_Level(NUMERIC)(1)(1) TLC_services(NUMERIC_ARRAY)(20)(0  0  0  0  0  0  0  0  0  0  0  0  0  0  0  0  0  0  0  0) Connection(NUMERIC_ARRAY)(20)(0  0  0  0  0  0  0  0  0  0  0  0  0  0  0  0  0  0  0  0) Dos_attack(NUMERIC)(1)(0) MITM_attack(NUMERIC)(1)(0) Virus_Attack(NUMERIC)(1)(0) Port_Scan_Attack(NUMERIC)(1)(0) Cyber_Fault(NUMERIC_ARRAY)(10)(0  0  0  0  0  0  0  0  0  0) Mechanical_Fault(NUMERIC)(1)(0) Conn_Fault(NUMERIC)(1)(0) TLC_revoke(NUMERIC_ARRAY)(20)(0  0  0  0  0  0  0  0  0  0  0  0  0  0  0  0  0  0  0  0)  *** OUTPUT RESOURCES *** NUM_OUTPUTS 4 TLC_CONN (20) TLC_SERVICE (20) CYBER_FAULT (10) MECH_FAULT (1), Parameter10=off, codeupdate=off, step_received=Connection=max(Connection_init,TLC_CONN); TLC_services=max(TLC_services_init,TLC_SERVICE); TLC_services=mod(TLC_services,10); TLC_revoke=floor(TLC_SERVICE/10);  Cyber_Fault=CYBER_FAULT;  Mechanical_Fault=max([Mechanical_Fault MECH_FAULT Mechanical_Fault_init]);  %TLC_services=TLC_services.*(1-TLC_revoke);  Operative_Level=1-Mechanical_Fault;, step_computed=, dynamic_computed=, step_sended=TLC_CONN=Connection*Operative_Level; TLC_SERVICE=TLC_services*Operative_Level+TLC_revoke*10;   CYBER_FAULT=Cyber_Fault*Operative_Level; MECH_FAULT=Mechanical_Fault;, id_entity=30, id_project=40, id_type=1, name_type=Optical_Wire, color=#99CCFF}
      mask prompts: Parameter1 "entity name"; Parameter2 "sampling time"; Parameter3 "project"; resources "input resources and state variables"; Parameter10 "Bring state variables to output"; codeupdate "update code from mask"
      mask help: This is a level-2 MATLAB file S-function which demonstrates CISIA entity
      mask DialogControl Container1 Prompt: All parameters
      mask Display: image('Icons/Optical_Wire.png')
  Wire_10b (31) : M-S-Function  FunctionName=cisia_msfun  Parameters=Parameter1, Parameter2, Parameter3, resources, Parameter10, codeupdate, step_received, step_computed, dynamic_computed, step_sended, id_entity, id_project, id_type, name_type, color  mask(S-function:msfcn_unit_delay){Parameter1='Wire_10b', Parameter2=1, Parameter3='ORO', resources=*** INPUT RESOURCES *** NUM_INPUTS 4 TLC_CONN (20) TLC_SERVICE (20) CYBER_FAULT (10) MECH_FAULT (1)  *** STATE VARIABLES *** NUM_VARIABLES 11 Operative_Level(NUMERIC)(1)(1) TLC_services(NUMERIC_ARRAY)(20)(0  0  0  0  0  0  0  0  0  0  0  0  0  0  0  0  0  0  0  0) Connection(NUMERIC_ARRAY)(20)(0  0  0  0  0  0  0  0  0  0  0  0  0  0  0  0  0  0  0  0) Dos_attack(NUMERIC)(1)(0) MITM_attack(NUMERIC)(1)(0) Virus_Attack(NUMERIC)(1)(0) Port_Scan_Attack(NUMERIC)(1)(0) Cyber_Fault(NUMERIC_ARRAY)(10)(0  0  0  0  0  0  0  0  0  0) Mechanical_Fault(NUMERIC)(1)(0) Conn_Fault(NUMERIC)(1)(0) TLC_revoke(NUMERIC_ARRAY)(20)(0  0  0  0  0  0  0  0  0  0  0  0  0  0  0  0  0  0  0  0)  *** OUTPUT RESOURCES *** NUM_OUTPUTS 4 TLC_CONN (20) TLC_SERVICE (20) CYBER_FAULT (10) MECH_FAULT (1), Parameter10=off, codeupdate=off, step_received=Connection=max(Connection_init,TLC_CONN); TLC_services=max(TLC_services_init,TLC_SERVICE); TLC_services=mod(TLC_services,10); TLC_revoke=floor(TLC_SERVICE/10);  Cyber_Fault=CYBER_FAULT;  Mechanical_Fault=max([Mechanical_Fault MECH_FAULT Mechanical_Fault_init]);  %TLC_services=TLC_services.*(1-TLC_revoke);  Operative_Level=1-Mechanical_Fault;, step_computed=, dynamic_computed=, step_sended=TLC_CONN=Connection*Operative_Level; TLC_SERVICE=TLC_services*Operative_Level+TLC_revoke*10;   CYBER_FAULT=Cyber_Fault*Operative_Level; MECH_FAULT=Mechanical_Fault;, id_entity=31, id_project=40, id_type=1, name_type=Optical_Wire, color=#99CCFF}
      mask prompts: Parameter1 "entity name"; Parameter2 "sampling time"; Parameter3 "project"; resources "input resources and state variables"; Parameter10 "Bring state variables to output"; codeupdate "update code from mask"
      mask help: This is a level-2 MATLAB file S-function which demonstrates CISIA entity
      mask DialogControl Container1 Prompt: All parameters
      mask Display: image('Icons/Optical_Wire.png')
  Wire_14 (42) : M-S-Function  FunctionName=cisia_msfun  Parameters=Parameter1, Parameter2, Parameter3, resources, Parameter10, codeupdate, step_received, step_computed, dynamic_computed, step_sended, id_entity, id_project, id_type, name_type, color  mask(S-function:msfcn_unit_delay){Parameter1='Wire_14', Parameter2=1, Parameter3='ORO', resources=*** INPUT RESOURCES *** NUM_INPUTS 4 TLC_CONN (20) TLC_SERVICE (20) CYBER_FAULT (10) MECH_FAULT (1)  *** STATE VARIABLES *** NUM_VARIABLES 11 Operative_Level(NUMERIC)(1)(1) TLC_services(NUMERIC_ARRAY)(20)(0  0  0  0  0  0  0  0  0  0  0  0  0  0  0  0  0  0  0  0) Connection(NUMERIC_ARRAY)(20)(0  0  0  0  0  0  0  0  0  0  0  0  0  0  0  0  0  0  0  0) Dos_attack(NUMERIC)(1)(0) MITM_attack(NUMERIC)(1)(0) Virus_Attack(NUMERIC)(1)(0) Port_Scan_Attack(NUMERIC)(1)(0) Cyber_Fault(NUMERIC_ARRAY)(10)(0  0  0  0  0  0  0  0  0  0) Mechanical_Fault(NUMERIC)(1)(0) Conn_Fault(NUMERIC)(1)(0) TLC_revoke(NUMERIC_ARRAY)(20)(0  0  0  0  0  0  0  0  0  0  0  0  0  0  0  0  0  0  0  0)  *** OUTPUT RESOURCES *** NUM_OUTPUTS 4 TLC_CONN (20) TLC_SERVICE (20) CYBER_FAULT (10) MECH_FAULT (1), Parameter10=off, codeupdate=off, step_received=Connection=max(Connection_init,TLC_CONN); TLC_services=max(TLC_services_init,TLC_SERVICE); TLC_services=mod(TLC_services,10); TLC_revoke=floor(TLC_SERVICE/10);  Cyber_Fault=CYBER_FAULT;  Mechanical_Fault=max([Mechanical_Fault MECH_FAULT Mechanical_Fault_init]);  %TLC_services=TLC_services.*(1-TLC_revoke);  Operative_Level=1-Mechanical_Fault;, step_computed=, dynamic_computed=, step_sended=TLC_CONN=Connection*Operative_Level; TLC_SERVICE=TLC_services*Operative_Level+TLC_revoke*10;   CYBER_FAULT=Cyber_Fault*Operative_Level; MECH_FAULT=Mechanical_Fault;, id_entity=42, id_project=40, id_type=1, name_type=Optical_Wire, color=#99CCFF}
      mask prompts: Parameter1 "entity name"; Parameter2 "sampling time"; Parameter3 "project"; resources "input resources and state variables"; Parameter10 "Bring state variables to output"; codeupdate "update code from mask"
      mask help: This is a level-2 MATLAB file S-function which demonstrates CISIA entity
      mask DialogControl Container1 Prompt: All parameters
      mask Display: image('Icons/Optical_Wire.png')
  Wire_14b (43) : M-S-Function  FunctionName=cisia_msfun  Parameters=Parameter1, Parameter2, Parameter3, resources, Parameter10, codeupdate, step_received, step_computed, dynamic_computed, step_sended, id_entity, id_project, id_type, name_type, color  mask(S-function:msfcn_unit_delay){Parameter1='Wire_14b', Parameter2=1, Parameter3='ORO', resources=*** INPUT RESOURCES *** NUM_INPUTS 4 TLC_CONN (20) TLC_SERVICE (20) CYBER_FAULT (10) MECH_FAULT (1)  *** STATE VARIABLES *** NUM_VARIABLES 11 Operative_Level(NUMERIC)(1)(1) TLC_services(NUMERIC_ARRAY)(20)(0  0  0  0  0  0  0  0  0  0  0  0  0  0  0  0  0  0  0  0) Connection(NUMERIC_ARRAY)(20)(0  0  0  0  0  0  0  0  0  0  0  0  0  0  0  0  0  0  0  0) Dos_attack(NUMERIC)(1)(0) MITM_attack(NUMERIC)(1)(0) Virus_Attack(NUMERIC)(1)(0) Port_Scan_Attack(NUMERIC)(1)(0) Cyber_Fault(NUMERIC_ARRAY)(10)(0  0  0  0  0  0  0  0  0  0) Mechanical_Fault(NUMERIC)(1)(0) Conn_Fault(NUMERIC)(1)(0) TLC_revoke(NUMERIC_ARRAY)(20)(0  0  0  0  0  0  0  0  0  0  0  0  0  0  0  0  0  0  0  0)  *** OUTPUT RESOURCES *** NUM_OUTPUTS 4 TLC_CONN (20) TLC_SERVICE (20) CYBER_FAULT (10) MECH_FAULT (1), Parameter10=off, codeupdate=off, step_received=Connection=max(Connection_init,TLC_CONN); TLC_services=max(TLC_services_init,TLC_SERVICE); TLC_services=mod(TLC_services,10); TLC_revoke=floor(TLC_SERVICE/10);  Cyber_Fault=CYBER_FAULT;  Mechanical_Fault=max([Mechanical_Fault MECH_FAULT Mechanical_Fault_init]);  %TLC_services=TLC_services.*(1-TLC_revoke);  Operative_Level=1-Mechanical_Fault;, step_computed=, dynamic_computed=, step_sended=TLC_CONN=Connection*Operative_Level; TLC_SERVICE=TLC_services*Operative_Level+TLC_revoke*10;   CYBER_FAULT=Cyber_Fault*Operative_Level; MECH_FAULT=Mechanical_Fault;, id_entity=43, id_project=40, id_type=1, name_type=Optical_Wire, color=#99CCFF}
      mask prompts: Parameter1 "entity name"; Parameter2 "sampling time"; Parameter3 "project"; resources "input resources and state variables"; Parameter10 "Bring state variables to output"; codeupdate "update code from mask"
      mask help: This is a level-2 MATLAB file S-function which demonstrates CISIA entity
      mask DialogControl Container1 Prompt: All parameters
      mask Display: image('Icons/Optical_Wire.png')
  Wire_16 (45) : M-S-Function  FunctionName=cisia_msfun  Parameters=Parameter1, Parameter2, Parameter3, resources, Parameter10, codeupdate, step_received, step_computed, dynamic_computed, step_sended, id_entity, id_project, id_type, name_type, color  mask(S-function:msfcn_unit_delay){Parameter1='Wire_16', Parameter2=1, Parameter3='ORO', resources=*** INPUT RESOURCES *** NUM_INPUTS 4 TLC_CONN (20) TLC_SERVICE (20) CYBER_FAULT (10) MECH_FAULT (1)  *** STATE VARIABLES *** NUM_VARIABLES 11 Operative_Level(NUMERIC)(1)(1) TLC_services(NUMERIC_ARRAY)(20)(0  0  0  0  0  0  0  0  0  0  0  0  0  0  0  0  0  0  0  0) Connection(NUMERIC_ARRAY)(20)(0  0  0  0  0  0  0  0  0  0  0  0  0  0  0  0  0  0  0  0) Dos_attack(NUMERIC)(1)(0) MITM_attack(NUMERIC)(1)(0) Virus_Attack(NUMERIC)(1)(0) Port_Scan_Attack(NUMERIC)(1)(0) Cyber_Fault(NUMERIC_ARRAY)(10)(0  0  0  0  0  0  0  0  0  0) Mechanical_Fault(NUMERIC)(1)(0) Conn_Fault(NUMERIC)(1)(0) TLC_revoke(NUMERIC_ARRAY)(20)(0  0  0  0  0  0  0  0  0  0  0  0  0  0  0  0  0  0  0  0)  *** OUTPUT RESOURCES *** NUM_OUTPUTS 4 TLC_CONN (20) TLC_SERVICE (20) CYBER_FAULT (10) MECH_FAULT (1), Parameter10=off, codeupdate=off, step_received=Connection=max(Connection_init,TLC_CONN); TLC_services=max(TLC_services_init,TLC_SERVICE); TLC_services=mod(TLC_services,10); TLC_revoke=floor(TLC_SERVICE/10);  Cyber_Fault=CYBER_FAULT;  Mechanical_Fault=max([Mechanical_Fault MECH_FAULT Mechanical_Fault_init]);  %TLC_services=TLC_services.*(1-TLC_revoke);  Operative_Level=1-Mechanical_Fault;, step_computed=, dynamic_computed=, step_sended=TLC_CONN=Connection*Operative_Level; TLC_SERVICE=TLC_services*Operative_Level+TLC_revoke*10;   CYBER_FAULT=Cyber_Fault*Operative_Level; MECH_FAULT=Mechanical_Fault;, id_entity=45, id_project=40, id_type=1, name_type=Optical_Wire, color=#99CCFF}
      mask prompts: Parameter1 "entity name"; Parameter2 "sampling time"; Parameter3 "project"; resources "input resources and state variables"; Parameter10 "Bring state variables to output"; codeupdate "update code from mask"
      mask help: This is a level-2 MATLAB file S-function which demonstrates CISIA entity
      mask DialogControl Container1 Prompt: All parameters
      mask Display: image('Icons/Optical_Wire.png')
  Wire_16a (50) : M-S-Function  FunctionName=cisia_msfun  Parameters=Parameter1, Parameter2, Parameter3, resources, Parameter10, codeupdate, step_received, step_computed, dynamic_computed, step_sended, id_entity, id_project, id_type, name_type, color  mask(S-function:msfcn_unit_delay){Parameter1='Wire_16a', Parameter2=1, Parameter3='ORO', resources=*** INPUT RESOURCES *** NUM_INPUTS 4 TLC_CONN (20) TLC_SERVICE (20) CYBER_FAULT (10) MECH_FAULT (1)  *** STATE VARIABLES *** NUM_VARIABLES 11 Operative_Level(NUMERIC)(1)(1) TLC_services(NUMERIC_ARRAY)(20)(0  0  0  0  0  0  0  0  0  0  0  0  0  0  0  0  0  0  0  0) Connection(NUMERIC_ARRAY)(20)(0  0  0  0  0  0  0  0  0  0  0  0  0  0  0  0  0  0  0  0) Dos_attack(NUMERIC)(1)(0) MITM_attack(NUMERIC)(1)(0) Virus_Attack(NUMERIC)(1)(0) Port_Scan_Attack(NUMERIC)(1)(0) Cyber_Fault(NUMERIC_ARRAY)(10)(0  0  0  0  0  0  0  0  0  0) Mechanical_Fault(NUMERIC)(1)(0) Conn_Fault(NUMERIC)(1)(0) TLC_revoke(NUMERIC_ARRAY)(20)(0  0  0  0  0  0  0  0  0  0  0  0  0  0  0  0  0  0  0  0)  *** OUTPUT RESOURCES *** NUM_OUTPUTS 4 TLC_CONN (20) TLC_SERVICE (20) CYBER_FAULT (10) MECH_FAULT (1), Parameter10=off, codeupdate=off, step_received=Connection=max(Connection_init,TLC_CONN); TLC_services=max(TLC_services_init,TLC_SERVICE); TLC_services=mod(TLC_services,10); TLC_revoke=floor(TLC_SERVICE/10);  Cyber_Fault=CYBER_FAULT;  Mechanical_Fault=max([Mechanical_Fault MECH_FAULT Mechanical_Fault_init]);  %TLC_services=TLC_services.*(1-TLC_revoke);  Operative_Level=1-Mechanical_Fault;, step_computed=, dynamic_computed=, step_sended=TLC_CONN=Connection*Operative_Level; TLC_SERVICE=TLC_services*Operative_Level+TLC_revoke*10;   CYBER_FAULT=Cyber_Fault*Operative_Level; MECH_FAULT=Mechanical_Fault;, id_entity=50, id_project=40, id_type=1, name_type=Optical_Wire, color=#99CCFF}
      mask prompts: Parameter1 "entity name"; Parameter2 "sampling time"; Parameter3 "project"; resources "input resources and state variables"; Parameter10 "Bring state variables to output"; codeupdate "update code from mask"
      mask help: This is a level-2 MATLAB file S-function which demonstrates CISIA entity
      mask DialogControl Container1 Prompt: All parameters
      mask Display: image('Icons/Optical_Wire.png')
  Wire_3 (11) : M-S-Function  FunctionName=cisia_msfun  Parameters=Parameter1, Parameter2, Parameter3, resources, Parameter10, codeupdate, step_received, step_computed, dynamic_computed, step_sended, id_entity, id_project, id_type, name_type, color  mask(S-function:msfcn_unit_delay){Parameter1='Wire_3', Parameter2=1, Parameter3='ORO', resources=*** INPUT RESOURCES *** NUM_INPUTS 4 TLC_CONN (20) TLC_SERVICE (20) CYBER_FAULT (10) MECH_FAULT (1)  *** STATE VARIABLES *** NUM_VARIABLES 11 Operative_Level(NUMERIC)(1)(1) TLC_services(NUMERIC_ARRAY)(20)(0  0  0  0  0  0  0  0  0  0  0  0  0  0  0  0  0  0  0  0) Connection(NUMERIC_ARRAY)(20)(0  0  0  0  0  0  0  0  0  0  0  0  0  0  0  0  0  0  0  0) Dos_attack(NUMERIC)(1)(0) MITM_attack(NUMERIC)(1)(0) Virus_Attack(NUMERIC)(1)(0) Port_Scan_Attack(NUMERIC)(1)(0) Cyber_Fault(NUMERIC_ARRAY)(10)(0  0  0  0  0  0  0  0  0  0) Mechanical_Fault(NUMERIC)(1)(0) Conn_Fault(NUMERIC)(1)(0) TLC_revoke(NUMERIC_ARRAY)(20)(0  0  0  0  0  0  0  0  0  0  0  0  0  0  0  0  0  0  0  0)  *** OUTPUT RESOURCES *** NUM_OUTPUTS 4 TLC_CONN (20) TLC_SERVICE (20) CYBER_FAULT (10) MECH_FAULT (1), Parameter10=off, codeupdate=off, step_received=Connection=max(Connection_init,TLC_CONN); TLC_services=max(TLC_services_init,TLC_SERVICE); TLC_services=mod(TLC_services,10); TLC_revoke=floor(TLC_SERVICE/10);  Cyber_Fault=CYBER_FAULT;  Mechanical_Fault=max([Mechanical_Fault MECH_FAULT Mechanical_Fault_init]);  %TLC_services=TLC_services.*(1-TLC_revoke);  Operative_Level=1-Mechanical_Fault;, step_computed=, dynamic_computed=, step_sended=TLC_CONN=Connection*Operative_Level; TLC_SERVICE=TLC_services*Operative_Level+TLC_revoke*10;   CYBER_FAULT=Cyber_Fault*Operative_Level; MECH_FAULT=Mechanical_Fault;, id_entity=11, id_project=40, id_type=1, name_type=Optical_Wire, color=#99CCFF}
      mask prompts: Parameter1 "entity name"; Parameter2 "sampling time"; Parameter3 "project"; resources "input resources and state variables"; Parameter10 "Bring state variables to output"; codeupdate "update code from mask"
      mask help: This is a level-2 MATLAB file S-function which demonstrates CISIA entity
      mask DialogControl Container1 Prompt: All parameters
      mask Display: image('Icons/Optical_Wire.png')
  Wire_3b (14) : M-S-Function  FunctionName=cisia_msfun  Parameters=Parameter1, Parameter2, Parameter3, resources, Parameter10, codeupdate, step_received, step_computed, dynamic_computed, step_sended, id_entity, id_project, id_type, name_type, color  mask(S-function:msfcn_unit_delay){Parameter1='Wire_3b', Parameter2=1, Parameter3='ORO', resources=*** INPUT RESOURCES *** NUM_INPUTS 4 TLC_CONN (20) TLC_SERVICE (20) CYBER_FAULT (10) MECH_FAULT (1)  *** STATE VARIABLES *** NUM_VARIABLES 11 Operative_Level(NUMERIC)(1)(1) TLC_services(NUMERIC_ARRAY)(20)(0  0  0  0  0  0  0  0  0  0  0  0  0  0  0  0  0  0  0  0) Connection(NUMERIC_ARRAY)(20)(0  0  0  0  0  0  0  0  0  0  0  0  0  0  0  0  0  0  0  0) Dos_attack(NUMERIC)(1)(0) MITM_attack(NUMERIC)(1)(0) Virus_Attack(NUMERIC)(1)(0) Port_Scan_Attack(NUMERIC)(1)(0) Cyber_Fault(NUMERIC_ARRAY)(10)(0  0  0  0  0  0  0  0  0  0) Mechanical_Fault(NUMERIC)(1)(0) Conn_Fault(NUMERIC)(1)(0) TLC_revoke(NUMERIC_ARRAY)(20)(0  0  0  0  0  0  0  0  0  0  0  0  0  0  0  0  0  0  0  0)  *** OUTPUT RESOURCES *** NUM_OUTPUTS 4 TLC_CONN (20) TLC_SERVICE (20) CYBER_FAULT (10) MECH_FAULT (1), Parameter10=off, codeupdate=off, step_received=Connection=max(Connection_init,TLC_CONN); TLC_services=max(TLC_services_init,TLC_SERVICE); TLC_services=mod(TLC_services,10); TLC_revoke=floor(TLC_SERVICE/10);  Cyber_Fault=CYBER_FAULT;  Mechanical_Fault=max([Mechanical_Fault MECH_FAULT Mechanical_Fault_init]);  %TLC_services=TLC_services.*(1-TLC_revoke);  Operative_Level=1-Mechanical_Fault;, step_computed=, dynamic_computed=, step_sended=TLC_CONN=Connection*Operative_Level; TLC_SERVICE=TLC_services*Operative_Level+TLC_revoke*10;   CYBER_FAULT=Cyber_Fault*Operative_Level; MECH_FAULT=Mechanical_Fault;, id_entity=14, id_project=40, id_type=1, name_type=Optical_Wire, color=#99CCFF}
      mask prompts: Parameter1 "entity name"; Parameter2 "sampling time"; Parameter3 "project"; resources "input resources and state variables"; Parameter10 "Bring state variables to output"; codeupdate "update code from mask"
      mask help: This is a level-2 MATLAB file S-function which demonstrates CISIA entity
      mask DialogControl Container1 Prompt: All parameters
      mask Display: image('Icons/Optical_Wire.png')
  Wire_4 (12) : M-S-Function  FunctionName=cisia_msfun  Parameters=Parameter1, Parameter2, Parameter3, resources, Parameter10, codeupdate, step_received, step_computed, dynamic_computed, step_sended, id_entity, id_project, id_type, name_type, color  mask(S-function:msfcn_unit_delay){Parameter1='Wire_4', Parameter2=1, Parameter3='ORO', resources=*** INPUT RESOURCES *** NUM_INPUTS 4 TLC_CONN (20) TLC_SERVICE (20) CYBER_FAULT (10) MECH_FAULT (1)  *** STATE VARIABLES *** NUM_VARIABLES 11 Operative_Level(NUMERIC)(1)(1) TLC_services(NUMERIC_ARRAY)(20)(0  0  0  0  0  0  0  0  0  0  0  0  0  0  0  0  0  0  0  0) Connection(NUMERIC_ARRAY)(20)(0  0  0  0  0  0  0  0  0  0  0  0  0  0  0  0  0  0  0  0) Dos_attack(NUMERIC)(1)(0) MITM_attack(NUMERIC)(1)(0) Virus_Attack(NUMERIC)(1)(0) Port_Scan_Attack(NUMERIC)(1)(0) Cyber_Fault(NUMERIC_ARRAY)(10)(0  0  0  0  0  0  0  0  0  0) Mechanical_Fault(NUMERIC)(1)(0) Conn_Fault(NUMERIC)(1)(0) TLC_revoke(NUMERIC_ARRAY)(20)(0  0  0  0  0  0  0  0  0  0  0  0  0  0  0  0  0  0  0  0)  *** OUTPUT RESOURCES *** NUM_OUTPUTS 4 TLC_CONN (20) TLC_SERVICE (20) CYBER_FAULT (10) MECH_FAULT (1), Parameter10=off, codeupdate=off, step_received=Connection=max(Connection_init,TLC_CONN); TLC_services=max(TLC_services_init,TLC_SERVICE); TLC_services=mod(TLC_services,10); TLC_revoke=floor(TLC_SERVICE/10);  Cyber_Fault=CYBER_FAULT;  Mechanical_Fault=max([Mechanical_Fault MECH_FAULT Mechanical_Fault_init]);  %TLC_services=TLC_services.*(1-TLC_revoke);  Operative_Level=1-Mechanical_Fault;, step_computed=, dynamic_computed=, step_sended=TLC_CONN=Connection*Operative_Level; TLC_SERVICE=TLC_services*Operative_Level+TLC_revoke*10;   CYBER_FAULT=Cyber_Fault*Operative_Level; MECH_FAULT=Mechanical_Fault;, id_entity=12, id_project=40, id_type=1, name_type=Optical_Wire, color=#99CCFF}
      mask prompts: Parameter1 "entity name"; Parameter2 "sampling time"; Parameter3 "project"; resources "input resources and state variables"; Parameter10 "Bring state variables to output"; codeupdate "update code from mask"
      mask help: This is a level-2 MATLAB file S-function which demonstrates CISIA entity
      mask DialogControl Container1 Prompt: All parameters
      mask Display: image('Icons/Optical_Wire.png')
  Wire_4b (13) : M-S-Function  FunctionName=cisia_msfun  Parameters=Parameter1, Parameter2, Parameter3, resources, Parameter10, codeupdate, step_received, step_computed, dynamic_computed, step_sended, id_entity, id_project, id_type, name_type, color  mask(S-function:msfcn_unit_delay){Parameter1='Wire_4b', Parameter2=1, Parameter3='ORO', resources=*** INPUT RESOURCES *** NUM_INPUTS 4 TLC_CONN (20) TLC_SERVICE (20) CYBER_FAULT (10) MECH_FAULT (1)  *** STATE VARIABLES *** NUM_VARIABLES 11 Operative_Level(NUMERIC)(1)(1) TLC_services(NUMERIC_ARRAY)(20)(0  0  0  0  0  0  0  0  0  0  0  0  0  0  0  0  0  0  0  0) Connection(NUMERIC_ARRAY)(20)(0  0  0  0  0  0  0  0  0  0  0  0  0  0  0  0  0  0  0  0) Dos_attack(NUMERIC)(1)(0) MITM_attack(NUMERIC)(1)(0) Virus_Attack(NUMERIC)(1)(0) Port_Scan_Attack(NUMERIC)(1)(0) Cyber_Fault(NUMERIC_ARRAY)(10)(0  0  0  0  0  0  0  0  0  0) Mechanical_Fault(NUMERIC)(1)(0) Conn_Fault(NUMERIC)(1)(0) TLC_revoke(NUMERIC_ARRAY)(20)(0  0  0  0  0  0  0  0  0  0  0  0  0  0  0  0  0  0  0  0)  *** OUTPUT RESOURCES *** NUM_OUTPUTS 4 TLC_CONN (20) TLC_SERVICE (20) CYBER_FAULT (10) MECH_FAULT (1), Parameter10=off, codeupdate=off, step_received=Connection=max(Connection_init,TLC_CONN); TLC_services=max(TLC_services_init,TLC_SERVICE); TLC_services=mod(TLC_services,10); TLC_revoke=floor(TLC_SERVICE/10);  Cyber_Fault=CYBER_FAULT;  Mechanical_Fault=max([Mechanical_Fault MECH_FAULT Mechanical_Fault_init]);  %TLC_services=TLC_services.*(1-TLC_revoke);  Operative_Level=1-Mechanical_Fault;, step_computed=, dynamic_computed=, step_sended=TLC_CONN=Connection*Operative_Level; TLC_SERVICE=TLC_services*Operative_Level+TLC_revoke*10;   CYBER_FAULT=Cyber_Fault*Operative_Level; MECH_FAULT=Mechanical_Fault;, id_entity=13, id_project=40, id_type=1, name_type=Optical_Wire, color=#99CCFF}
      mask prompts: Parameter1 "entity name"; Parameter2 "sampling time"; Parameter3 "project"; resources "input resources and state variables"; Parameter10 "Bring state variables to output"; codeupdate "update code from mask"
      mask help: This is a level-2 MATLAB file S-function which demonstrates CISIA entity
      mask DialogControl Container1 Prompt: All parameters
      mask Display: image('Icons/Optical_Wire.png')
  Wire_5 (15) : M-S-Function  FunctionName=cisia_msfun  Parameters=Parameter1, Parameter2, Parameter3, resources, Parameter10, codeupdate, step_received, step_computed, dynamic_computed, step_sended, id_entity, id_project, id_type, name_type, color  mask(S-function:msfcn_unit_delay){Parameter1='Wire_5', Parameter2=1, Parameter3='ORO', resources=*** INPUT RESOURCES *** NUM_INPUTS 4 TLC_CONN (20) TLC_SERVICE (20) CYBER_FAULT (10) MECH_FAULT (1)  *** STATE VARIABLES *** NUM_VARIABLES 11 Operative_Level(NUMERIC)(1)(1) TLC_services(NUMERIC_ARRAY)(20)(0  0  0  0  0  0  0  0  0  0  0  0  0  0  0  0  0  0  0  0) Connection(NUMERIC_ARRAY)(20)(0  0  0  0  0  0  0  0  0  0  0  0  0  0  0  0  0  0  0  0) Dos_attack(NUMERIC)(1)(0) MITM_attack(NUMERIC)(1)(0) Virus_Attack(NUMERIC)(1)(0) Port_Scan_Attack(NUMERIC)(1)(0) Cyber_Fault(NUMERIC_ARRAY)(10)(0  0  0  0  0  0  0  0  0  0) Mechanical_Fault(NUMERIC)(1)(0) Conn_Fault(NUMERIC)(1)(0) TLC_revoke(NUMERIC_ARRAY)(20)(0  0  0  0  0  0  0  0  0  0  0  0  0  0  0  0  0  0  0  0)  *** OUTPUT RESOURCES *** NUM_OUTPUTS 4 TLC_CONN (20) TLC_SERVICE (20) CYBER_FAULT (10) MECH_FAULT (1), Parameter10=off, codeupdate=off, step_received=Connection=max(Connection_init,TLC_CONN); TLC_services=max(TLC_services_init,TLC_SERVICE); TLC_services=mod(TLC_services,10); TLC_revoke=floor(TLC_SERVICE/10);  Cyber_Fault=CYBER_FAULT;  Mechanical_Fault=max([Mechanical_Fault MECH_FAULT Mechanical_Fault_init]);  %TLC_services=TLC_services.*(1-TLC_revoke);  Operative_Level=1-Mechanical_Fault;, step_computed=, dynamic_computed=, step_sended=TLC_CONN=Connection*Operative_Level; TLC_SERVICE=TLC_services*Operative_Level+TLC_revoke*10;   CYBER_FAULT=Cyber_Fault*Operative_Level; MECH_FAULT=Mechanical_Fault;, id_entity=15, id_project=40, id_type=1, name_type=Optical_Wire, color=#99CCFF}
      mask prompts: Parameter1 "entity name"; Parameter2 "sampling time"; Parameter3 "project"; resources "input resources and state variables"; Parameter10 "Bring state variables to output"; codeupdate "update code from mask"
      mask help: This is a level-2 MATLAB file S-function which demonstrates CISIA entity
      mask DialogControl Container1 Prompt: All parameters
      mask Display: image('Icons/Optical_Wire.png')
  Wire_5b (16) : M-S-Function  FunctionName=cisia_msfun  Parameters=Parameter1, Parameter2, Parameter3, resources, Parameter10, codeupdate, step_received, step_computed, dynamic_computed, step_sended, id_entity, id_project, id_type, name_type, color  mask(S-function:msfcn_unit_delay){Parameter1='Wire_5b', Parameter2=1, Parameter3='ORO', resources=*** INPUT RESOURCES *** NUM_INPUTS 4 TLC_CONN (20) TLC_SERVICE (20) CYBER_FAULT (10) MECH_FAULT (1)  *** STATE VARIABLES *** NUM_VARIABLES 11 Operative_Level(NUMERIC)(1)(1) TLC_services(NUMERIC_ARRAY)(20)(0  0  0  0  0  0  0  0  0  0  0  0  0  0  0  0  0  0  0  0) Connection(NUMERIC_ARRAY)(20)(0  0  0  0  0  0  0  0  0  0  0  0  0  0  0  0  0  0  0  0) Dos_attack(NUMERIC)(1)(0) MITM_attack(NUMERIC)(1)(0) Virus_Attack(NUMERIC)(1)(0) Port_Scan_Attack(NUMERIC)(1)(0) Cyber_Fault(NUMERIC_ARRAY)(10)(0  0  0  0  0  0  0  0  0  0) Mechanical_Fault(NUMERIC)(1)(0) Conn_Fault(NUMERIC)(1)(0) TLC_revoke(NUMERIC_ARRAY)(20)(0  0  0  0  0  0  0  0  0  0  0  0  0  0  0  0  0  0  0  0)  *** OUTPUT RESOURCES *** NUM_OUTPUTS 4 TLC_CONN (20) TLC_SERVICE (20) CYBER_FAULT (10) MECH_FAULT (1), Parameter10=off, codeupdate=off, step_received=Connection=max(Connection_init,TLC_CONN); TLC_services=max(TLC_services_init,TLC_SERVICE); TLC_services=mod(TLC_services,10); TLC_revoke=floor(TLC_SERVICE/10);  Cyber_Fault=CYBER_FAULT;  Mechanical_Fault=max([Mechanical_Fault MECH_FAULT Mechanical_Fault_init]);  %TLC_services=TLC_services.*(1-TLC_revoke);  Operative_Level=1-Mechanical_Fault;, step_computed=, dynamic_computed=, step_sended=TLC_CONN=Connection*Operative_Level; TLC_SERVICE=TLC_services*Operative_Level+TLC_revoke*10;   CYBER_FAULT=Cyber_Fault*Operative_Level; MECH_FAULT=Mechanical_Fault;, id_entity=16, id_project=40, id_type=1, name_type=Optical_Wire, color=#99CCFF}
      mask prompts: Parameter1 "entity name"; Parameter2 "sampling time"; Parameter3 "project"; resources "input resources and state variables"; Parameter10 "Bring state variables to output"; codeupdate "update code from mask"
      mask help: This is a level-2 MATLAB file S-function which demonstrates CISIA entity
      mask DialogControl Container1 Prompt: All parameters
      mask Display: image('Icons/Optical_Wire.png')
  Wire_6 (17) : M-S-Function  FunctionName=cisia_msfun  Parameters=Parameter1, Parameter2, Parameter3, resources, Parameter10, codeupdate, step_received, step_computed, dynamic_computed, step_sended, id_entity, id_project, id_type, name_type, color  mask(S-function:msfcn_unit_delay){Parameter1='Wire_6', Parameter2=1, Parameter3='ORO', resources=*** INPUT RESOURCES *** NUM_INPUTS 4 TLC_CONN (20) TLC_SERVICE (20) CYBER_FAULT (10) MECH_FAULT (1)  *** STATE VARIABLES *** NUM_VARIABLES 11 Operative_Level(NUMERIC)(1)(1) TLC_services(NUMERIC_ARRAY)(20)(0  0  0  0  0  0  0  0  0  0  0  0  0  0  0  0  0  0  0  0) Connection(NUMERIC_ARRAY)(20)(0  0  0  0  0  0  0  0  0  0  0  0  0  0  0  0  0  0  0  0) Dos_attack(NUMERIC)(1)(0) MITM_attack(NUMERIC)(1)(0) Virus_Attack(NUMERIC)(1)(0) Port_Scan_Attack(NUMERIC)(1)(0) Cyber_Fault(NUMERIC_ARRAY)(10)(0  0  0  0  0  0  0  0  0  0) Mechanical_Fault(NUMERIC)(1)(0) Conn_Fault(NUMERIC)(1)(0) TLC_revoke(NUMERIC_ARRAY)(20)(0  0  0  0  0  0  0  0  0  0  0  0  0  0  0  0  0  0  0  0)  *** OUTPUT RESOURCES *** NUM_OUTPUTS 4 TLC_CONN (20) TLC_SERVICE (20) CYBER_FAULT (10) MECH_FAULT (1), Parameter10=off, codeupdate=off, step_received=Connection=max(Connection_init,TLC_CONN); TLC_services=max(TLC_services_init,TLC_SERVICE); TLC_services=mod(TLC_services,10); TLC_revoke=floor(TLC_SERVICE/10);  Cyber_Fault=CYBER_FAULT;  Mechanical_Fault=max([Mechanical_Fault MECH_FAULT Mechanical_Fault_init]);  %TLC_services=TLC_services.*(1-TLC_revoke);  Operative_Level=1-Mechanical_Fault;, step_computed=, dynamic_computed=, step_sended=TLC_CONN=Connection*Operative_Level; TLC_SERVICE=TLC_services*Operative_Level+TLC_revoke*10;   CYBER_FAULT=Cyber_Fault*Operative_Level; MECH_FAULT=Mechanical_Fault;, id_entity=17, id_project=40, id_type=1, name_type=Optical_Wire, color=#99CCFF}
      mask prompts: Parameter1 "entity name"; Parameter2 "sampling time"; Parameter3 "project"; resources "input resources and state variables"; Parameter10 "Bring state variables to output"; codeupdate "update code from mask"
      mask help: This is a level-2 MATLAB file S-function which demonstrates CISIA entity
      mask DialogControl Container1 Prompt: All parameters
      mask Display: image('Icons/Optical_Wire.png')
  Wire_6b (18) : M-S-Function  FunctionName=cisia_msfun  Parameters=Parameter1, Parameter2, Parameter3, resources, Parameter10, codeupdate, step_received, step_computed, dynamic_computed, step_sended, id_entity, id_project, id_type, name_type, color  mask(S-function:msfcn_unit_delay){Parameter1='Wire_6b', Parameter2=1, Parameter3='ORO', resources=*** INPUT RESOURCES *** NUM_INPUTS 4 TLC_CONN (20) TLC_SERVICE (20) CYBER_FAULT (10) MECH_FAULT (1)  *** STATE VARIABLES *** NUM_VARIABLES 11 Operative_Level(NUMERIC)(1)(1) TLC_services(NUMERIC_ARRAY)(20)(0  0  0  0  0  0  0  0  0  0  0  0  0  0  0  0  0  0  0  0) Connection(NUMERIC_ARRAY)(20)(0  0  0  0  0  0  0  0  0  0  0  0  0  0  0  0  0  0  0  0) Dos_attack(NUMERIC)(1)(0) MITM_attack(NUMERIC)(1)(0) Virus_Attack(NUMERIC)(1)(0) Port_Scan_Attack(NUMERIC)(1)(0) Cyber_Fault(NUMERIC_ARRAY)(10)(0  0  0  0  0  0  0  0  0  0) Mechanical_Fault(NUMERIC)(1)(0) Conn_Fault(NUMERIC)(1)(0) TLC_revoke(NUMERIC_ARRAY)(20)(0  0  0  0  0  0  0  0  0  0  0  0  0  0  0  0  0  0  0  0)  *** OUTPUT RESOURCES *** NUM_OUTPUTS 4 TLC_CONN (20) TLC_SERVICE (20) CYBER_FAULT (10) MECH_FAULT (1), Parameter10=off, codeupdate=off, step_received=Connection=max(Connection_init,TLC_CONN); TLC_services=max(TLC_services_init,TLC_SERVICE); TLC_services=mod(TLC_services,10); TLC_revoke=floor(TLC_SERVICE/10);  Cyber_Fault=CYBER_FAULT;  Mechanical_Fault=max([Mechanical_Fault MECH_FAULT Mechanical_Fault_init]);  %TLC_services=TLC_services.*(1-TLC_revoke);  Operative_Level=1-Mechanical_Fault;, step_computed=, dynamic_computed=, step_sended=TLC_CONN=Connection*Operative_Level; TLC_SERVICE=TLC_services*Operative_Level+TLC_revoke*10;   CYBER_FAULT=Cyber_Fault*Operative_Level; MECH_FAULT=Mechanical_Fault;, id_entity=18, id_project=40, id_type=1, name_type=Optical_Wire, color=#99CCFF}
      mask prompts: Parameter1 "entity name"; Parameter2 "sampling time"; Parameter3 "project"; resources "input resources and state variables"; Parameter10 "Bring state variables to output"; codeupdate "update code from mask"
      mask help: This is a level-2 MATLAB file S-function which demonstrates CISIA entity
      mask DialogControl Container1 Prompt: All parameters
      mask Display: image('Icons/Optical_Wire.png')
  Wire_7 (19) : M-S-Function  FunctionName=cisia_msfun  Parameters=Parameter1, Parameter2, Parameter3, resources, Parameter10, codeupdate, step_received, step_computed, dynamic_computed, step_sended, id_entity, id_project, id_type, name_type, color  mask(S-function:msfcn_unit_delay){Parameter1='Wire_7', Parameter2=1, Parameter3='ORO', resources=*** INPUT RESOURCES *** NUM_INPUTS 4 TLC_CONN (20) TLC_SERVICE (20) CYBER_FAULT (10) MECH_FAULT (1)  *** STATE VARIABLES *** NUM_VARIABLES 11 Operative_Level(NUMERIC)(1)(1) TLC_services(NUMERIC_ARRAY)(20)(0  0  0  0  0  0  0  0  0  0  0  0  0  0  0  0  0  0  0  0) Connection(NUMERIC_ARRAY)(20)(0  0  0  0  0  0  0  0  0  0  0  0  0  0  0  0  0  0  0  0) Dos_attack(NUMERIC)(1)(0) MITM_attack(NUMERIC)(1)(0) Virus_Attack(NUMERIC)(1)(0) Port_Scan_Attack(NUMERIC)(1)(0) Cyber_Fault(NUMERIC_ARRAY)(10)(0  0  0  0  0  0  0  0  0  0) Mechanical_Fault(NUMERIC)(1)(0) Conn_Fault(NUMERIC)(1)(0) TLC_revoke(NUMERIC_ARRAY)(20)(0  0  0  0  0  0  0  0  0  0  0  0  0  0  0  0  0  0  0  0)  *** OUTPUT RESOURCES *** NUM_OUTPUTS 4 TLC_CONN (20) TLC_SERVICE (20) CYBER_FAULT (10) MECH_FAULT (1), Parameter10=off, codeupdate=off, step_received=Connection=max(Connection_init,TLC_CONN); TLC_services=max(TLC_services_init,TLC_SERVICE); TLC_services=mod(TLC_services,10); TLC_revoke=floor(TLC_SERVICE/10);  Cyber_Fault=CYBER_FAULT;  Mechanical_Fault=max([Mechanical_Fault MECH_FAULT Mechanical_Fault_init]);  %TLC_services=TLC_services.*(1-TLC_revoke);  Operative_Level=1-Mechanical_Fault;, step_computed=, dynamic_computed=, step_sended=TLC_CONN=Connection*Operative_Level; TLC_SERVICE=TLC_services*Operative_Level+TLC_revoke*10;   CYBER_FAULT=Cyber_Fault*Operative_Level; MECH_FAULT=Mechanical_Fault;, id_entity=19, id_project=40, id_type=1, name_type=Optical_Wire, color=#99CCFF}
      mask prompts: Parameter1 "entity name"; Parameter2 "sampling time"; Parameter3 "project"; resources "input resources and state variables"; Parameter10 "Bring state variables to output"; codeupdate "update code from mask"
      mask help: This is a level-2 MATLAB file S-function which demonstrates CISIA entity
      mask DialogControl Container1 Prompt: All parameters
      mask Display: image('Icons/Optical_Wire.png')
  Wire_7b (20) : M-S-Function  FunctionName=cisia_msfun  Parameters=Parameter1, Parameter2, Parameter3, resources, Parameter10, codeupdate, step_received, step_computed, dynamic_computed, step_sended, id_entity, id_project, id_type, name_type, color  mask(S-function:msfcn_unit_delay){Parameter1='Wire_7b', Parameter2=1, Parameter3='ORO', resources=*** INPUT RESOURCES *** NUM_INPUTS 4 TLC_CONN (20) TLC_SERVICE (20) CYBER_FAULT (10) MECH_FAULT (1)  *** STATE VARIABLES *** NUM_VARIABLES 11 Operative_Level(NUMERIC)(1)(1) TLC_services(NUMERIC_ARRAY)(20)(0  0  0  0  0  0  0  0  0  0  0  0  0  0  0  0  0  0  0  0) Connection(NUMERIC_ARRAY)(20)(0  0  0  0  0  0  0  0  0  0  0  0  0  0  0  0  0  0  0  0) Dos_attack(NUMERIC)(1)(0) MITM_attack(NUMERIC)(1)(0) Virus_Attack(NUMERIC)(1)(0) Port_Scan_Attack(NUMERIC)(1)(0) Cyber_Fault(NUMERIC_ARRAY)(10)(0  0  0  0  0  0  0  0  0  0) Mechanical_Fault(NUMERIC)(1)(0) Conn_Fault(NUMERIC)(1)(0) TLC_revoke(NUMERIC_ARRAY)(20)(0  0  0  0  0  0  0  0  0  0  0  0  0  0  0  0  0  0  0  0)  *** OUTPUT RESOURCES *** NUM_OUTPUTS 4 TLC_CONN (20) TLC_SERVICE (20) CYBER_FAULT (10) MECH_FAULT (1), Parameter10=off, codeupdate=off, step_received=Connection=max(Connection_init,TLC_CONN); TLC_services=max(TLC_services_init,TLC_SERVICE); TLC_services=mod(TLC_services,10); TLC_revoke=floor(TLC_SERVICE/10);  Cyber_Fault=CYBER_FAULT;  Mechanical_Fault=max([Mechanical_Fault MECH_FAULT Mechanical_Fault_init]);  %TLC_services=TLC_services.*(1-TLC_revoke);  Operative_Level=1-Mechanical_Fault;, step_computed=, dynamic_computed=, step_sended=TLC_CONN=Connection*Operative_Level; TLC_SERVICE=TLC_services*Operative_Level+TLC_revoke*10;   CYBER_FAULT=Cyber_Fault*Operative_Level; MECH_FAULT=Mechanical_Fault;, id_entity=20, id_project=40, id_type=1, name_type=Optical_Wire, color=#99CCFF}
      mask prompts: Parameter1 "entity name"; Parameter2 "sampling time"; Parameter3 "project"; resources "input resources and state variables"; Parameter10 "Bring state variables to output"; codeupdate "update code from mask"
      mask help: This is a level-2 MATLAB file S-function which demonstrates CISIA entity
      mask DialogControl Container1 Prompt: All parameters
      mask Display: image('Icons/Optical_Wire.png')
  Wire_8 (21) : M-S-Function  FunctionName=cisia_msfun  Parameters=Parameter1, Parameter2, Parameter3, resources, Parameter10, codeupdate, step_received, step_computed, dynamic_computed, step_sended, id_entity, id_project, id_type, name_type, color  mask(S-function:msfcn_unit_delay){Parameter1='Wire_8', Parameter2=1, Parameter3='ORO', resources=*** INPUT RESOURCES *** NUM_INPUTS 4 TLC_CONN (20) TLC_SERVICE (20) CYBER_FAULT (10) MECH_FAULT (1)  *** STATE VARIABLES *** NUM_VARIABLES 11 Operative_Level(NUMERIC)(1)(1) TLC_services(NUMERIC_ARRAY)(20)(0  0  0  0  0  0  0  0  0  0  0  0  0  0  0  0  0  0  0  0) Connection(NUMERIC_ARRAY)(20)(0  0  0  0  0  0  0  0  0  0  0  0  0  0  0  0  0  0  0  0) Dos_attack(NUMERIC)(1)(0) MITM_attack(NUMERIC)(1)(0) Virus_Attack(NUMERIC)(1)(0) Port_Scan_Attack(NUMERIC)(1)(0) Cyber_Fault(NUMERIC_ARRAY)(10)(0  0  0  0  0  0  0  0  0  0) Mechanical_Fault(NUMERIC)(1)(0) Conn_Fault(NUMERIC)(1)(0) TLC_revoke(NUMERIC_ARRAY)(20)(0  0  0  0  0  0  0  0  0  0  0  0  0  0  0  0  0  0  0  0)  *** OUTPUT RESOURCES *** NUM_OUTPUTS 4 TLC_CONN (20) TLC_SERVICE (20) CYBER_FAULT (10) MECH_FAULT (1), Parameter10=off, codeupdate=off, step_received=Connection=max(Connection_init,TLC_CONN); TLC_services=max(TLC_services_init,TLC_SERVICE); TLC_services=mod(TLC_services,10); TLC_revoke=floor(TLC_SERVICE/10);  Cyber_Fault=CYBER_FAULT;  Mechanical_Fault=max([Mechanical_Fault MECH_FAULT Mechanical_Fault_init]);  %TLC_services=TLC_services.*(1-TLC_revoke);  Operative_Level=1-Mechanical_Fault;, step_computed=, dynamic_computed=, step_sended=TLC_CONN=Connection*Operative_Level; TLC_SERVICE=TLC_services*Operative_Level+TLC_revoke*10;   CYBER_FAULT=Cyber_Fault*Operative_Level; MECH_FAULT=Mechanical_Fault;, id_entity=21, id_project=40, id_type=1, name_type=Optical_Wire, color=#99CCFF}
      mask prompts: Parameter1 "entity name"; Parameter2 "sampling time"; Parameter3 "project"; resources "input resources and state variables"; Parameter10 "Bring state variables to output"; codeupdate "update code from mask"
      mask help: This is a level-2 MATLAB file S-function which demonstrates CISIA entity
      mask DialogControl Container1 Prompt: All parameters
      mask Display: image('Icons/Optical_Wire.png')
  Wire_8b (22) : M-S-Function  FunctionName=cisia_msfun  Parameters=Parameter1, Parameter2, Parameter3, resources, Parameter10, codeupdate, step_received, step_computed, dynamic_computed, step_sended, id_entity, id_project, id_type, name_type, color  mask(S-function:msfcn_unit_delay){Parameter1='Wire_8b', Parameter2=1, Parameter3='ORO', resources=*** INPUT RESOURCES *** NUM_INPUTS 4 TLC_CONN (20) TLC_SERVICE (20) CYBER_FAULT (10) MECH_FAULT (1)  *** STATE VARIABLES *** NUM_VARIABLES 11 Operative_Level(NUMERIC)(1)(1) TLC_services(NUMERIC_ARRAY)(20)(0  0  0  0  0  0  0  0  0  0  0  0  0  0  0  0  0  0  0  0) Connection(NUMERIC_ARRAY)(20)(0  0  0  0  0  0  0  0  0  0  0  0  0  0  0  0  0  0  0  0) Dos_attack(NUMERIC)(1)(0) MITM_attack(NUMERIC)(1)(0) Virus_Attack(NUMERIC)(1)(0) Port_Scan_Attack(NUMERIC)(1)(0) Cyber_Fault(NUMERIC_ARRAY)(10)(0  0  0  0  0  0  0  0  0  0) Mechanical_Fault(NUMERIC)(1)(0) Conn_Fault(NUMERIC)(1)(0) TLC_revoke(NUMERIC_ARRAY)(20)(0  0  0  0  0  0  0  0  0  0  0  0  0  0  0  0  0  0  0  0)  *** OUTPUT RESOURCES *** NUM_OUTPUTS 4 TLC_CONN (20) TLC_SERVICE (20) CYBER_FAULT (10) MECH_FAULT (1), Parameter10=off, codeupdate=off, step_received=Connection=max(Connection_init,TLC_CONN); TLC_services=max(TLC_services_init,TLC_SERVICE); TLC_services=mod(TLC_services,10); TLC_revoke=floor(TLC_SERVICE/10);  Cyber_Fault=CYBER_FAULT;  Mechanical_Fault=max([Mechanical_Fault MECH_FAULT Mechanical_Fault_init]);  %TLC_services=TLC_services.*(1-TLC_revoke);  Operative_Level=1-Mechanical_Fault;, step_computed=, dynamic_computed=, step_sended=TLC_CONN=Connection*Operative_Level; TLC_SERVICE=TLC_services*Operative_Level+TLC_revoke*10;   CYBER_FAULT=Cyber_Fault*Operative_Level; MECH_FAULT=Mechanical_Fault;, id_entity=22, id_project=40, id_type=1, name_type=Optical_Wire, color=#99CCFF}
      mask prompts: Parameter1 "entity name"; Parameter2 "sampling time"; Parameter3 "project"; resources "input resources and state variables"; Parameter10 "Bring state variables to output"; codeupdate "update code from mask"
      mask help: This is a level-2 MATLAB file S-function which demonstrates CISIA entity
      mask DialogControl Container1 Prompt: All parameters
      mask Display: image('Icons/Optical_Wire.png')
  media2 : MATLAB Function  TreatAsAtomicUnit=on
  media3 : MATLAB Function  TreatAsAtomicUnit=on
  media4 : MATLAB Function  TreatAsAtomicUnit=on
  media9 : MATLAB Function  TreatAsAtomicUnit=on
  tag scope: POWER_1=global
  wires:
  Nex_3 (92)/1 -> TLC_conn4/1, R_Wire_1b (99)/1, TLC_conn3/1, Wire_8 (21)/1  "TLC_CONN"
  R_Wire_1b (99)/1 -> TLC_conn1/1  "TLC_CONN"
  TLC_conn1/1 -> Nex_4 (93)/1  "TLC_CONN"
  ASR9006_3 (87)/3 -> Wire_16 (45)/3, Wire_6b (18)/3  "CYBER_FAULT"
  Wire_8 (21)/2 -> ASR920_3 (85)/2  "TLC_SERVICE"
  ASR920_3 (85)/3 -> Wire_8b (22)/3  "CYBER_FAULT"
  ASR9006_3 (87)/1 -> Wire_16 (45)/1, Wire_6b (18)/1  "TLC_CONN"
  Wire_8b (22)/4 -> Wire_8 (21)/4  "MECH_FAULT"
  Wire_8 (21)/1 -> ASR920_3 (85)/1  "TLC_CONN"
  Wire_8 (21)/3 -> ASR920_3 (85)/3  "CYBER_FAULT"
  Wire_4 (12)/2 -> ASR903_3 (89)/2  "TLC_SERVICE"
  Wire_6 (17)/4 -> Wire_6b (18)/4  "MECH_FAULT"
  ASR920_3 (85)/2 -> Wire_8b (22)/2  "TLC_SERVICE"
  Wire_8 (21)/4 -> Wire_8b (22)/4  "MECH_FAULT"
  Wire_4 (12)/3 -> ASR903_3 (89)/3  "CYBER_FAULT"
  ASR903_3 (89)/1 -> Wire_10 (30)/1, Wire_4b (13)/1  "TLC_CONN"
  Wire_4 (12)/1 -> ASR903_3 (89)/1  "TLC_CONN"
  ASR920_3 (85)/1 -> Wire_8b (22)/1  "TLC_CONN"
  ASR903_3 (89)/3 -> Wire_10 (30)/3, Wire_4b (13)/3  "CYBER_FAULT"
  ASR903_3 (89)/2 -> Wire_10 (30)/2, Wire_4b (13)/2  "TLC_SERVICE"
  Wire_10 (30)/4 -> Wire_10b (31)/4  "MECH_FAULT"
  Nex_3 (92)/3 -> CYBER_fault3/1, R_Wire_1b (99)/3, Wire_8 (21)/3, CYBER_fault1/1  "CYBER_FAULT"
  TLC_conn2/1 -> Nex_3 (92)/1  "TLC_CONN"
  TLC_service2/1 -> Nex_3 (92)/2  "TLC_SERVICE"
  CYBER_fault2/1 -> Nex_3 (92)/3  "CYBER_FAULT"
  TLC_conn3/1 -> Wire_4 (12)/1  "TLC_CONN"
  TLC_service3/1 -> Wire_4 (12)/2  "TLC_SERVICE"
  CYBER_fault1/1 -> Wire_4 (12)/3  "CYBER_FAULT"
  Wire_10b (31)/1 -> TLC_conn3/2  "TLC_CONN"
  Wire_10b (31)/2 -> TLC_service3/2  "TLC_SERVICE"
  Wire_10b (31)/3 -> CYBER_fault1/2  "CYBER_FAULT"
  Wire_4b (13)/4 -> Wire_4 (12)/4  "MECH_FAULT"
  Wire_4 (12)/4 -> Wire_4b (13)/4  "MECH_FAULT"
  Wire_10b (31)/4 -> Wire_10 (30)/4  "MECH_FAULT"
  Wire_8b (22)/1 -> TLC_conn2/2  "TLC_CONN"
  Wire_4b (13)/1 -> TLC_conn2/3  "TLC_CONN"
  Wire_6b (18)/1 -> TLC_conn2/4  "TLC_CONN"
  Wire_8b (22)/2 -> TLC_service2/2  "TLC_SERVICE"
  Wire_4b (13)/2 -> TLC_service2/3  "TLC_SERVICE"
  Wire_6b (18)/2 -> TLC_service2/4  "TLC_SERVICE"
  Wire_6b (18)/3 -> CYBER_fault2/4  "CYBER_FAULT"
  Wire_4b (13)/3 -> CYBER_fault2/3  "CYBER_FAULT"
  Wire_8b (22)/3 -> CYBER_fault2/2  "CYBER_FAULT"
  R_Wire_1 (98)/1 -> TLC_conn2/1  "TLC_CONN"
  R_Wire_1 (98)/2 -> TLC_service2/1  "TLC_SERVICE"
  R_Wire_1 (98)/3 -> CYBER_fault2/1  "CYBER_FAULT"
  R_Wire_1 (98)/4 -> R_Wire_1b (99)/4  "MECH_FAULT"
  R_Wire_1b (99)/4 -> R_Wire_1 (98)/4  "MECH_FAULT"
  ASR9006_3 (87)/2 -> ROUTE_AL_3 (5)/1  "TLC_SERVICE"
  ROUTE_AL_3 (5)/1 -> Wire_6b (18)/2  "TLC_SERVICE"
  Wire_16 (45)/1 -> OLT_1 (25)/1  "TLC_CONN"
  Wire_16 (45)/2 -> Display/1, OLT_1 (25)/2  "TLC_SERVICE"
  Wire_16 (45)/3 -> OLT_1 (25)/3  "CYBER_FAULT"
  OLT_1 (25)/1 -> Wire_16a (50)/1  "TLC_CONN"
  OLT_1 (25)/2 -> Splitter_1 (54)/1, Wire_16a (50)/2  "TLC_SERVICE"
  OLT_1 (25)/3 -> Splitter_1 (54)/2, Wire_16a (50)/3  "CYBER_FAULT"
  Wire_16 (45)/4 -> Wire_16a (50)/4  "MECH_FAULT"
  Wire_16a (50)/4 -> Wire_16 (45)/4  "MECH_FAULT"
  TLC_conn4/1 -> Wire_6 (17)/1  "TLC_CONN"
  TLC_service4/1 -> Wire_6 (17)/2  "TLC_SERVICE"
  CYBER_fault3/1 -> Wire_6 (17)/3  "CYBER_FAULT"
  Wire_16a (50)/1 -> TLC_conn4/2  "TLC_CONN"
  Wire_16a (50)/2 -> TLC_service4/2  "TLC_SERVICE"
  Wire_16a (50)/3 -> CYBER_fault3/2  "CYBER_FAULT"
  ROUTE_AL_3 (5)/2 -> Wire_16 (45)/2  "TLC_SERVICE"
  ONU_1 (55)/1 -> ANTENNA_1 (56)/1  "TLC_SERVICE"
  R_Wire_1b (99)/2 -> TLC_service1/1  "TLC_SERVICE"
  R_Wire_1b (99)/3 -> "CYBER_fault1 "/1  "CYBER_FAULT"
  Nex_4 (93)/2 -> ROUTE_AL_2 (4)/1  "TLC_SERVICE"
  TLC_service1/1 -> Nex_4 (93)/2  "TLC_SERVICE"
  "CYBER_fault1 "/1 -> Nex_4 (93)/3  "CYBER_FAULT"
  ONU_2 (58)/1 -> ANTENNA_2 (60)/1  "TLC_SERVICE"
  ROUTE_AL_4 (6)/2 -> Wire_14 (42)/2  "TLC_SERVICE"
  ROUTE_AL_4 (6)/1 -> Wire_3b (14)/2  "TLC_SERVICE"
  ASR9006_4 (88)/1 -> Wire_14 (42)/1, Wire_3b (14)/1  "TLC_CONN"
  ASR9006_4 (88)/2 -> ROUTE_AL_4 (6)/1  "TLC_SERVICE"
  ASR9006_4 (88)/3 -> Wire_14 (42)/3, Wire_3b (14)/3  "CYBER_FAULT"
  TLC_service5/1 -> Wire_3 (11)/2  "TLC_SERVICE"
  TLC_conn5/1 -> Wire_3 (11)/1  "TLC_CONN"
  CYBER_fault4/1 -> Wire_3 (11)/3  "CYBER_FAULT"
  Wire_14 (42)/1 -> OLT_2 (57)/1  "TLC_CONN"
  Wire_14 (42)/2 -> OLT_2 (57)/2  "TLC_SERVICE"
  Wire_14 (42)/3 -> OLT_2 (57)/3  "CYBER_FAULT"
  OLT_2 (57)/1 -> Wire_14b (43)/1  "TLC_CONN"
  OLT_2 (57)/2 -> Splitter_2 (59)/1, Wire_14b (43)/2  "TLC_SERVICE"
  OLT_2 (57)/3 -> Splitter_2 (59)/2, Wire_14b (43)/3  "CYBER_FAULT"
  Wire_3 (11)/1 -> ASR9006_4 (88)/1  "TLC_CONN"
  Wire_3 (11)/2 -> ASR9006_4 (88)/2  "TLC_SERVICE"
  Wire_3 (11)/3 -> ASR9006_4 (88)/3  "CYBER_FAULT"
  Wire_14b (43)/1 -> TLC_conn5/2  "TLC_CONN"
  Wire_14b (43)/2 -> TLC_service5/2  "TLC_SERVICE"
  Wire_14b (43)/3 -> CYBER_fault4/2  "CYBER_FAULT"
  Nex_4 (93)/1 -> R_Wire_1 (98)/1, Wire_7 (19)/1, Wire_5 (15)/1, TLC_conn5/1  "TLC_CONN"
  ROUTE_AL_2 (4)/4 -> TLC_service5/1  "TLC_SERVICE"
  Nex_4 (93)/3 -> Wire_5 (15)/3, R_Wire_1 (98)/3, Wire_7 (19)/3, CYBER_fault4/1  "CYBER_FAULT"
  ROUTE_AL_2 (4)/3 -> Wire_5 (15)/2  "TLC_SERVICE"
  ROUTE_AL_2 (4)/2 -> Wire_7 (19)/2  "TLC_SERVICE"
  Wire_7 (19)/1 -> ASR903_4 (90)/1  "TLC_CONN"
  Wire_7 (19)/2 -> ASR903_4 (90)/2  "TLC_SERVICE"
  Wire_7 (19)/3 -> ASR903_4 (90)/3  "CYBER_FAULT"
  ASR903_4 (90)/1 -> Wire_7b (20)/1  "TLC_CONN"
  ASR903_4 (90)/2 -> Wire_7b (20)/2  "TLC_SERVICE"
  ASR903_4 (90)/3 -> Wire_7b (20)/3  "CYBER_FAULT"
  Wire_5 (15)/1 -> ASR920_4 (86)/1  "TLC_CONN"
  Wire_5 (15)/2 -> ASR920_4 (86)/2  "TLC_SERVICE"
  Wire_5 (15)/3 -> ASR920_4 (86)/3  "CYBER_FAULT"
  ASR920_4 (86)/1 -> Wire_5b (16)/1  "TLC_CONN"
  ASR920_4 (86)/2 -> Wire_5b (16)/2  "TLC_SERVICE"
  ASR920_4 (86)/3 -> Wire_5b (16)/3  "CYBER_FAULT"
  Wire_7b (20)/4 -> Wire_7 (19)/4  "MECH_FAULT"
  Wire_7 (19)/4 -> Wire_7b (20)/4  "MECH_FAULT"
  Wire_5b (16)/4 -> Wire_5 (15)/4  "MECH_FAULT"
  Wire_5 (15)/4 -> Wire_5b (16)/4  "MECH_FAULT"
  Wire_7b (20)/1 -> TLC_conn1/2  "TLC_CONN"
  Wire_5b (16)/1 -> TLC_conn1/3  "TLC_CONN"
  Wire_3b (14)/1 -> TLC_conn1/4  "TLC_CONN"
  Wire_7b (20)/2 -> TLC_service1/2  "TLC_SERVICE"
  Wire_5b (16)/2 -> TLC_service1/3  "TLC_SERVICE"
  Wire_3b (14)/2 -> TLC_service1/4  "TLC_SERVICE"
  Wire_7b (20)/3 -> "CYBER_fault1 "/2  "CYBER_FAULT"
  Wire_5b (16)/3 -> "CYBER_fault1 "/3  "CYBER_FAULT"
  Wire_3b (14)/3 -> "CYBER_fault1 "/4  "CYBER_FAULT"
  Wire_3b (14)/4 -> Wire_3 (11)/4  "MECH_FAULT"
  Wire_3 (11)/4 -> Wire_3b (14)/4  "MECH_FAULT"
  Splitter_1 (54)/1 -> ONU_2 (58)/1  "TLC_SERVICE"
  Splitter_2 (59)/1 -> Display9/1, ONU_1 (55)/1  "TLC_SERVICE"
  ROUTE_AL_2 (4)/1 -> R_Wire_1 (98)/2  "TLC_SERVICE"
  OLT_2 (57)/4 -> Splitter_2 (59)/3  "NGPON_CONN"
  Splitter_2 (59)/2 -> ONU_1 (55)/2  "CYBER_FAULT"
  Splitter_2 (59)/3 -> Display1/1, ONU_1 (55)/4  "NGPON_CONN"
  Splitter_2 (59)/4 -> OLT_2 (57)/6  "NGPON_IN"
  ONU_1 (55)/2 -> ANTENNA_1 (56)/2  "CYBER_FAULT"
  ONU_1 (55)/3 -> ANTENNA_1 (56)/4  "NGPON_CONN"
  MOBILE1/1 -> Aveiro_Sea_Port (61)/1  "TLC_SERVICE"
  MOBILE2/1 -> Aveiro_Sea_Port (61)/2  "CYBER_FAULT"
  MOBILE3/1 -> Display5/1, Aveiro_Sea_Port (61)/3  "R_CONN"
  ANTENNA_1 (56)/1 -> MOBILE1/1  "TLC_SERVICE"
  ANTENNA_2 (60)/1 -> MOBILE1/2  "TLC_SERVICE"
  ANTENNA_1 (56)/2 -> MOBILE2/1  "CYBER_FAULT"
  ANTENNA_2 (60)/2 -> MOBILE2/2  "CYBER_FAULT"
  ANTENNA_1 (56)/3 -> MOBILE3/1  "R_CONN"
  ANTENNA_2 (60)/3 -> MOBILE3/2  "R_CONN"
  ONU_2 (58)/2 -> ANTENNA_2 (60)/2  "CYBER_FAULT"
  ONU_2 (58)/3 -> Display6/1, ANTENNA_2 (60)/4  "NGPON_CONN"
  Aveiro_Sea_Port (61)/1 -> Display2/1, MOBILE_1 (147)/1  "TLC_SERVICE"
  Aveiro_Sea_Port (61)/2 -> MOBILE_1 (147)/2  "CYBER_FAULT"
  Aveiro_Sea_Port (61)/3 -> Display10/1, MOBILE_1 (147)/3  "R_CONN"
